simulink model "EDoS_model"  (R2020b)
settings: Solver=VariableStepAuto  StartTime=0.0  StopTime=200000  RelTol=1e-3
values from neighbouring files (symbols this model uses):
  attackRate = 0    [init_model.m]
  initialLoopWaitTime = 1000    [init_model.m]    (also in plot_results.m = 50)
  lowerUtilThreshold = 50    [init_model.m]    (also in plot_results.m)
  maxCores = 35    [init_model.m]    (also in plot_results.m)
  routineRate = 4    [init_model.m]    (also in plot_results.m)
  scalingLoopDelay = 500    [init_model.m]    (also in plot_results.m = 5)
  scalingStep = 2    [init_model.m]    (also in plot_results.m)
  upperUtilThreshold = 80    [init_model.m]    (also in plot_results.m)
undefined symbols (not defined in the file or in its folder): m, n
libraries: simulink x2
(part 2 of 3)

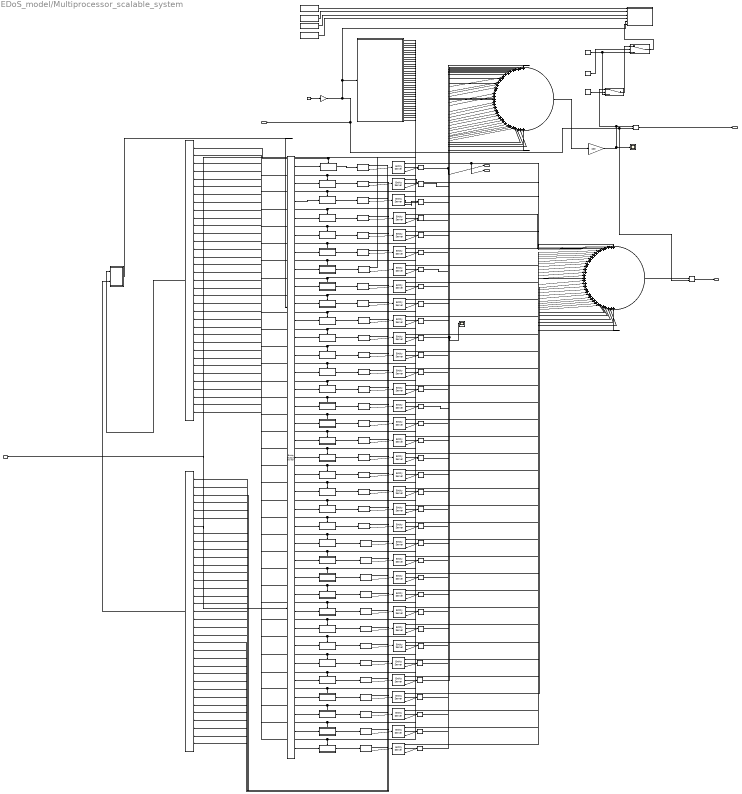
== system EDoS_model/Multiprocessor_scalable_system ==
  In1 : Inport
  Balancer : Subsystem
  Blocker : Subsystem
      settings: PortSchema="{\"entries\":[{\"content\":{\"sides\":[{\"content\":{\"connectorIds\":[\"In1\"]},\"type\":\"ConnectorPlacement.EquallySpacedRectSide\",\"uuid\":\"22857888-3c5c-4d01-b6fe-cd28fcf3e26a\"},{\"content\":{\"connectorIds\":[\"Out1\"],\"side\":\"RIGHT\"},\"type\":\"ConnectorPlacement.EquallySpacedRectSide\",\"uuid\":\"96f331b9-a29b-4997-ac5d-363cc8c82408\"},{\"content\":{\"connectorIds\":[\"In2\"],\"side\":\"TOP\"},\"type\":\"ConnectorPlacement.EquallySpacedRectSide\",\"uuid\":\"a53d43ab-ab12-479d-a738-753383dbd2f4\"},{\"content\":{\"connectorIds\":[],\"side\":\"HIDDEN\"},\"type\":\"ConnectorPlacement.EquallySpacedRectSide\",\"uuid\":\"fd9f22b1-3292-4974-90d3-70a5045257e9\"}]},\"type\":\"ConnectorPlacement.EquallySpacedConnector\",\"uuid\":\"b457ec3b-3668-4afe-a989-4fa0f92502cf\"}],\"packageUris\":[\"http://schema.mathworks.com/mf0/Connector/R2020b\"],\"version\":\"1.0\"}"
  Blocker1 : Subsystem
      settings: PortSchema="{\"entries\":[{\"content\":{\"sides\":[{\"content\":{\"connectorIds\":[\"In1\"]},\"type\":\"ConnectorPlacement.EquallySpacedRectSide\",\"uuid\":\"22857888-3c5c-4d01-b6fe-cd28fcf3e26a\"},{\"content\":{\"connectorIds\":[\"Out1\"],\"side\":\"RIGHT\"},\"type\":\"ConnectorPlacement.EquallySpacedRectSide\",\"uuid\":\"96f331b9-a29b-4997-ac5d-363cc8c82408\"},{\"content\":{\"connectorIds\":[\"In2\"],\"side\":\"TOP\"},\"type\":\"ConnectorPlacement.EquallySpacedRectSide\",\"uuid\":\"a53d43ab-ab12-479d-a738-753383dbd2f4\"},{\"content\":{\"connectorIds\":[],\"side\":\"HIDDEN\"},\"type\":\"ConnectorPlacement.EquallySpacedRectSide\",\"uuid\":\"fd9f22b1-3292-4974-90d3-70a5045257e9\"}]},\"type\":\"ConnectorPlacement.EquallySpacedConnector\",\"uuid\":\"b457ec3b-3668-4afe-a989-4fa0f92502cf\"}],\"packageUris\":[\"http://schema.mathworks.com/mf0/Connector/R2020b\"],\"version\":\"1.0\"}"
  Blocker10 : Subsystem
      settings: PortSchema="{\"entries\":[{\"content\":{\"sides\":[{\"content\":{\"connectorIds\":[\"In1\"]},\"type\":\"ConnectorPlacement.EquallySpacedRectSide\",\"uuid\":\"22857888-3c5c-4d01-b6fe-cd28fcf3e26a\"},{\"content\":{\"connectorIds\":[\"Out1\"],\"side\":\"RIGHT\"},\"type\":\"ConnectorPlacement.EquallySpacedRectSide\",\"uuid\":\"96f331b9-a29b-4997-ac5d-363cc8c82408\"},{\"content\":{\"connectorIds\":[\"In2\"],\"side\":\"TOP\"},\"type\":\"ConnectorPlacement.EquallySpacedRectSide\",\"uuid\":\"a53d43ab-ab12-479d-a738-753383dbd2f4\"},{\"content\":{\"connectorIds\":[],\"side\":\"HIDDEN\"},\"type\":\"ConnectorPlacement.EquallySpacedRectSide\",\"uuid\":\"fd9f22b1-3292-4974-90d3-70a5045257e9\"}]},\"type\":\"ConnectorPlacement.EquallySpacedConnector\",\"uuid\":\"b457ec3b-3668-4afe-a989-4fa0f92502cf\"}],\"packageUris\":[\"http://schema.mathworks.com/mf0/Connector/R2020b\"],\"version\":\"1.0\"}"
  Blocker11 : Subsystem
      settings: PortSchema="{\"entries\":[{\"content\":{\"sides\":[{\"content\":{\"connectorIds\":[\"In1\"]},\"type\":\"ConnectorPlacement.EquallySpacedRectSide\",\"uuid\":\"22857888-3c5c-4d01-b6fe-cd28fcf3e26a\"},{\"content\":{\"connectorIds\":[\"Out1\"],\"side\":\"RIGHT\"},\"type\":\"ConnectorPlacement.EquallySpacedRectSide\",\"uuid\":\"96f331b9-a29b-4997-ac5d-363cc8c82408\"},{\"content\":{\"connectorIds\":[\"In2\"],\"side\":\"TOP\"},\"type\":\"ConnectorPlacement.EquallySpacedRectSide\",\"uuid\":\"a53d43ab-ab12-479d-a738-753383dbd2f4\"},{\"content\":{\"connectorIds\":[],\"side\":\"HIDDEN\"},\"type\":\"ConnectorPlacement.EquallySpacedRectSide\",\"uuid\":\"fd9f22b1-3292-4974-90d3-70a5045257e9\"}]},\"type\":\"ConnectorPlacement.EquallySpacedConnector\",\"uuid\":\"b457ec3b-3668-4afe-a989-4fa0f92502cf\"}],\"packageUris\":[\"http://schema.mathworks.com/mf0/Connector/R2020b\"],\"version\":\"1.0\"}"
  Blocker12 : Subsystem
      settings: PortSchema="{\"entries\":[{\"content\":{\"sides\":[{\"content\":{\"connectorIds\":[\"In1\"]},\"type\":\"ConnectorPlacement.EquallySpacedRectSide\",\"uuid\":\"22857888-3c5c-4d01-b6fe-cd28fcf3e26a\"},{\"content\":{\"connectorIds\":[\"Out1\"],\"side\":\"RIGHT\"},\"type\":\"ConnectorPlacement.EquallySpacedRectSide\",\"uuid\":\"96f331b9-a29b-4997-ac5d-363cc8c82408\"},{\"content\":{\"connectorIds\":[\"In2\"],\"side\":\"TOP\"},\"type\":\"ConnectorPlacement.EquallySpacedRectSide\",\"uuid\":\"a53d43ab-ab12-479d-a738-753383dbd2f4\"},{\"content\":{\"connectorIds\":[],\"side\":\"HIDDEN\"},\"type\":\"ConnectorPlacement.EquallySpacedRectSide\",\"uuid\":\"fd9f22b1-3292-4974-90d3-70a5045257e9\"}]},\"type\":\"ConnectorPlacement.EquallySpacedConnector\",\"uuid\":\"b457ec3b-3668-4afe-a989-4fa0f92502cf\"}],\"packageUris\":[\"http://schema.mathworks.com/mf0/Connector/R2020b\"],\"version\":\"1.0\"}"
  Blocker13 : Subsystem
      settings: PortSchema="{\"entries\":[{\"content\":{\"sides\":[{\"content\":{\"connectorIds\":[\"In1\"]},\"type\":\"ConnectorPlacement.EquallySpacedRectSide\",\"uuid\":\"22857888-3c5c-4d01-b6fe-cd28fcf3e26a\"},{\"content\":{\"connectorIds\":[\"Out1\"],\"side\":\"RIGHT\"},\"type\":\"ConnectorPlacement.EquallySpacedRectSide\",\"uuid\":\"96f331b9-a29b-4997-ac5d-363cc8c82408\"},{\"content\":{\"connectorIds\":[\"In2\"],\"side\":\"TOP\"},\"type\":\"ConnectorPlacement.EquallySpacedRectSide\",\"uuid\":\"a53d43ab-ab12-479d-a738-753383dbd2f4\"},{\"content\":{\"connectorIds\":[],\"side\":\"HIDDEN\"},\"type\":\"ConnectorPlacement.EquallySpacedRectSide\",\"uuid\":\"fd9f22b1-3292-4974-90d3-70a5045257e9\"}]},\"type\":\"ConnectorPlacement.EquallySpacedConnector\",\"uuid\":\"b457ec3b-3668-4afe-a989-4fa0f92502cf\"}],\"packageUris\":[\"http://schema.mathworks.com/mf0/Connector/R2020b\"],\"version\":\"1.0\"}"
  Blocker14 : Subsystem
      settings: PortSchema="{\"entries\":[{\"content\":{\"sides\":[{\"content\":{\"connectorIds\":[\"In1\"]},\"type\":\"ConnectorPlacement.EquallySpacedRectSide\",\"uuid\":\"22857888-3c5c-4d01-b6fe-cd28fcf3e26a\"},{\"content\":{\"connectorIds\":[\"Out1\"],\"side\":\"RIGHT\"},\"type\":\"ConnectorPlacement.EquallySpacedRectSide\",\"uuid\":\"96f331b9-a29b-4997-ac5d-363cc8c82408\"},{\"content\":{\"connectorIds\":[\"In2\"],\"side\":\"TOP\"},\"type\":\"ConnectorPlacement.EquallySpacedRectSide\",\"uuid\":\"a53d43ab-ab12-479d-a738-753383dbd2f4\"},{\"content\":{\"connectorIds\":[],\"side\":\"HIDDEN\"},\"type\":\"ConnectorPlacement.EquallySpacedRectSide\",\"uuid\":\"fd9f22b1-3292-4974-90d3-70a5045257e9\"}]},\"type\":\"ConnectorPlacement.EquallySpacedConnector\",\"uuid\":\"b457ec3b-3668-4afe-a989-4fa0f92502cf\"}],\"packageUris\":[\"http://schema.mathworks.com/mf0/Connector/R2020b\"],\"version\":\"1.0\"}"
  Blocker15 : Subsystem
      settings: PortSchema="{\"entries\":[{\"content\":{\"sides\":[{\"content\":{\"connectorIds\":[\"In1\"]},\"type\":\"ConnectorPlacement.EquallySpacedRectSide\",\"uuid\":\"22857888-3c5c-4d01-b6fe-cd28fcf3e26a\"},{\"content\":{\"connectorIds\":[\"Out1\"],\"side\":\"RIGHT\"},\"type\":\"ConnectorPlacement.EquallySpacedRectSide\",\"uuid\":\"96f331b9-a29b-4997-ac5d-363cc8c82408\"},{\"content\":{\"connectorIds\":[\"In2\"],\"side\":\"TOP\"},\"type\":\"ConnectorPlacement.EquallySpacedRectSide\",\"uuid\":\"a53d43ab-ab12-479d-a738-753383dbd2f4\"},{\"content\":{\"connectorIds\":[],\"side\":\"HIDDEN\"},\"type\":\"ConnectorPlacement.EquallySpacedRectSide\",\"uuid\":\"fd9f22b1-3292-4974-90d3-70a5045257e9\"}]},\"type\":\"ConnectorPlacement.EquallySpacedConnector\",\"uuid\":\"b457ec3b-3668-4afe-a989-4fa0f92502cf\"}],\"packageUris\":[\"http://schema.mathworks.com/mf0/Connector/R2020b\"],\"version\":\"1.0\"}"
  Blocker16 : Subsystem
      settings: PortSchema="{\"entries\":[{\"content\":{\"sides\":[{\"content\":{\"connectorIds\":[\"In1\"]},\"type\":\"ConnectorPlacement.EquallySpacedRectSide\",\"uuid\":\"22857888-3c5c-4d01-b6fe-cd28fcf3e26a\"},{\"content\":{\"connectorIds\":[\"Out1\"],\"side\":\"RIGHT\"},\"type\":\"ConnectorPlacement.EquallySpacedRectSide\",\"uuid\":\"96f331b9-a29b-4997-ac5d-363cc8c82408\"},{\"content\":{\"connectorIds\":[\"In2\"],\"side\":\"TOP\"},\"type\":\"ConnectorPlacement.EquallySpacedRectSide\",\"uuid\":\"a53d43ab-ab12-479d-a738-753383dbd2f4\"},{\"content\":{\"connectorIds\":[],\"side\":\"HIDDEN\"},\"type\":\"ConnectorPlacement.EquallySpacedRectSide\",\"uuid\":\"fd9f22b1-3292-4974-90d3-70a5045257e9\"}]},\"type\":\"ConnectorPlacement.EquallySpacedConnector\",\"uuid\":\"b457ec3b-3668-4afe-a989-4fa0f92502cf\"}],\"packageUris\":[\"http://schema.mathworks.com/mf0/Connector/R2020b\"],\"version\":\"1.0\"}"
  Blocker17 : Subsystem
      settings: PortSchema="{\"entries\":[{\"content\":{\"sides\":[{\"content\":{\"connectorIds\":[\"In1\"]},\"type\":\"ConnectorPlacement.EquallySpacedRectSide\",\"uuid\":\"22857888-3c5c-4d01-b6fe-cd28fcf3e26a\"},{\"content\":{\"connectorIds\":[\"Out1\"],\"side\":\"RIGHT\"},\"type\":\"ConnectorPlacement.EquallySpacedRectSide\",\"uuid\":\"96f331b9-a29b-4997-ac5d-363cc8c82408\"},{\"content\":{\"connectorIds\":[\"In2\"],\"side\":\"TOP\"},\"type\":\"ConnectorPlacement.EquallySpacedRectSide\",\"uuid\":\"a53d43ab-ab12-479d-a738-753383dbd2f4\"},{\"content\":{\"connectorIds\":[],\"side\":\"HIDDEN\"},\"type\":\"ConnectorPlacement.EquallySpacedRectSide\",\"uuid\":\"fd9f22b1-3292-4974-90d3-70a5045257e9\"}]},\"type\":\"ConnectorPlacement.EquallySpacedConnector\",\"uuid\":\"b457ec3b-3668-4afe-a989-4fa0f92502cf\"}],\"packageUris\":[\"http://schema.mathworks.com/mf0/Connector/R2020b\"],\"version\":\"1.0\"}"
  Blocker18 : Subsystem
      settings: PortSchema="{\"entries\":[{\"content\":{\"sides\":[{\"content\":{\"connectorIds\":[\"In1\"]},\"type\":\"ConnectorPlacement.EquallySpacedRectSide\",\"uuid\":\"22857888-3c5c-4d01-b6fe-cd28fcf3e26a\"},{\"content\":{\"connectorIds\":[\"Out1\"],\"side\":\"RIGHT\"},\"type\":\"ConnectorPlacement.EquallySpacedRectSide\",\"uuid\":\"96f331b9-a29b-4997-ac5d-363cc8c82408\"},{\"content\":{\"connectorIds\":[\"In2\"],\"side\":\"TOP\"},\"type\":\"ConnectorPlacement.EquallySpacedRectSide\",\"uuid\":\"a53d43ab-ab12-479d-a738-753383dbd2f4\"},{\"content\":{\"connectorIds\":[],\"side\":\"HIDDEN\"},\"type\":\"ConnectorPlacement.EquallySpacedRectSide\",\"uuid\":\"fd9f22b1-3292-4974-90d3-70a5045257e9\"}]},\"type\":\"ConnectorPlacement.EquallySpacedConnector\",\"uuid\":\"b457ec3b-3668-4afe-a989-4fa0f92502cf\"}],\"packageUris\":[\"http://schema.mathworks.com/mf0/Connector/R2020b\"],\"version\":\"1.0\"}"
  Blocker19 : Subsystem
      settings: PortSchema="{\"entries\":[{\"content\":{\"sides\":[{\"content\":{\"connectorIds\":[\"In1\"]},\"type\":\"ConnectorPlacement.EquallySpacedRectSide\",\"uuid\":\"22857888-3c5c-4d01-b6fe-cd28fcf3e26a\"},{\"content\":{\"connectorIds\":[\"Out1\"],\"side\":\"RIGHT\"},\"type\":\"ConnectorPlacement.EquallySpacedRectSide\",\"uuid\":\"96f331b9-a29b-4997-ac5d-363cc8c82408\"},{\"content\":{\"connectorIds\":[\"In2\"],\"side\":\"TOP\"},\"type\":\"ConnectorPlacement.EquallySpacedRectSide\",\"uuid\":\"a53d43ab-ab12-479d-a738-753383dbd2f4\"},{\"content\":{\"connectorIds\":[],\"side\":\"HIDDEN\"},\"type\":\"ConnectorPlacement.EquallySpacedRectSide\",\"uuid\":\"fd9f22b1-3292-4974-90d3-70a5045257e9\"}]},\"type\":\"ConnectorPlacement.EquallySpacedConnector\",\"uuid\":\"b457ec3b-3668-4afe-a989-4fa0f92502cf\"}],\"packageUris\":[\"http://schema.mathworks.com/mf0/Connector/R2020b\"],\"version\":\"1.0\"}"
  Blocker2 : Subsystem
      settings: PortSchema="{\"entries\":[{\"content\":{\"sides\":[{\"content\":{\"connectorIds\":[\"In1\"]},\"type\":\"ConnectorPlacement.EquallySpacedRectSide\",\"uuid\":\"22857888-3c5c-4d01-b6fe-cd28fcf3e26a\"},{\"content\":{\"connectorIds\":[\"Out1\"],\"side\":\"RIGHT\"},\"type\":\"ConnectorPlacement.EquallySpacedRectSide\",\"uuid\":\"96f331b9-a29b-4997-ac5d-363cc8c82408\"},{\"content\":{\"connectorIds\":[\"In2\"],\"side\":\"TOP\"},\"type\":\"ConnectorPlacement.EquallySpacedRectSide\",\"uuid\":\"a53d43ab-ab12-479d-a738-753383dbd2f4\"},{\"content\":{\"connectorIds\":[],\"side\":\"HIDDEN\"},\"type\":\"ConnectorPlacement.EquallySpacedRectSide\",\"uuid\":\"fd9f22b1-3292-4974-90d3-70a5045257e9\"}]},\"type\":\"ConnectorPlacement.EquallySpacedConnector\",\"uuid\":\"b457ec3b-3668-4afe-a989-4fa0f92502cf\"}],\"packageUris\":[\"http://schema.mathworks.com/mf0/Connector/R2020b\"],\"version\":\"1.0\"}"
  Blocker20 : Subsystem
      settings: PortSchema="{\"entries\":[{\"content\":{\"sides\":[{\"content\":{\"connectorIds\":[\"In1\"]},\"type\":\"ConnectorPlacement.EquallySpacedRectSide\",\"uuid\":\"22857888-3c5c-4d01-b6fe-cd28fcf3e26a\"},{\"content\":{\"connectorIds\":[\"Out1\"],\"side\":\"RIGHT\"},\"type\":\"ConnectorPlacement.EquallySpacedRectSide\",\"uuid\":\"96f331b9-a29b-4997-ac5d-363cc8c82408\"},{\"content\":{\"connectorIds\":[\"In2\"],\"side\":\"TOP\"},\"type\":\"ConnectorPlacement.EquallySpacedRectSide\",\"uuid\":\"a53d43ab-ab12-479d-a738-753383dbd2f4\"},{\"content\":{\"connectorIds\":[],\"side\":\"HIDDEN\"},\"type\":\"ConnectorPlacement.EquallySpacedRectSide\",\"uuid\":\"fd9f22b1-3292-4974-90d3-70a5045257e9\"}]},\"type\":\"ConnectorPlacement.EquallySpacedConnector\",\"uuid\":\"b457ec3b-3668-4afe-a989-4fa0f92502cf\"}],\"packageUris\":[\"http://schema.mathworks.com/mf0/Connector/R2020b\"],\"version\":\"1.0\"}"
  Blocker21 : Subsystem
      settings: PortSchema="{\"entries\":[{\"content\":{\"sides\":[{\"content\":{\"connectorIds\":[\"In1\"]},\"type\":\"ConnectorPlacement.EquallySpacedRectSide\",\"uuid\":\"22857888-3c5c-4d01-b6fe-cd28fcf3e26a\"},{\"content\":{\"connectorIds\":[\"Out1\"],\"side\":\"RIGHT\"},\"type\":\"ConnectorPlacement.EquallySpacedRectSide\",\"uuid\":\"96f331b9-a29b-4997-ac5d-363cc8c82408\"},{\"content\":{\"connectorIds\":[\"In2\"],\"side\":\"TOP\"},\"type\":\"ConnectorPlacement.EquallySpacedRectSide\",\"uuid\":\"a53d43ab-ab12-479d-a738-753383dbd2f4\"},{\"content\":{\"connectorIds\":[],\"side\":\"HIDDEN\"},\"type\":\"ConnectorPlacement.EquallySpacedRectSide\",\"uuid\":\"fd9f22b1-3292-4974-90d3-70a5045257e9\"}]},\"type\":\"ConnectorPlacement.EquallySpacedConnector\",\"uuid\":\"b457ec3b-3668-4afe-a989-4fa0f92502cf\"}],\"packageUris\":[\"http://schema.mathworks.com/mf0/Connector/R2020b\"],\"version\":\"1.0\"}"
  Blocker22 : Subsystem
      settings: PortSchema="{\"entries\":[{\"content\":{\"sides\":[{\"content\":{\"connectorIds\":[\"In1\"]},\"type\":\"ConnectorPlacement.EquallySpacedRectSide\",\"uuid\":\"22857888-3c5c-4d01-b6fe-cd28fcf3e26a\"},{\"content\":{\"connectorIds\":[\"Out1\"],\"side\":\"RIGHT\"},\"type\":\"ConnectorPlacement.EquallySpacedRectSide\",\"uuid\":\"96f331b9-a29b-4997-ac5d-363cc8c82408\"},{\"content\":{\"connectorIds\":[\"In2\"],\"side\":\"TOP\"},\"type\":\"ConnectorPlacement.EquallySpacedRectSide\",\"uuid\":\"a53d43ab-ab12-479d-a738-753383dbd2f4\"},{\"content\":{\"connectorIds\":[],\"side\":\"HIDDEN\"},\"type\":\"ConnectorPlacement.EquallySpacedRectSide\",\"uuid\":\"fd9f22b1-3292-4974-90d3-70a5045257e9\"}]},\"type\":\"ConnectorPlacement.EquallySpacedConnector\",\"uuid\":\"b457ec3b-3668-4afe-a989-4fa0f92502cf\"}],\"packageUris\":[\"http://schema.mathworks.com/mf0/Connector/R2020b\"],\"version\":\"1.0\"}"
  Blocker23 : Subsystem
      settings: PortSchema="{\"entries\":[{\"content\":{\"sides\":[{\"content\":{\"connectorIds\":[\"In1\"]},\"type\":\"ConnectorPlacement.EquallySpacedRectSide\",\"uuid\":\"22857888-3c5c-4d01-b6fe-cd28fcf3e26a\"},{\"content\":{\"connectorIds\":[\"Out1\"],\"side\":\"RIGHT\"},\"type\":\"ConnectorPlacement.EquallySpacedRectSide\",\"uuid\":\"96f331b9-a29b-4997-ac5d-363cc8c82408\"},{\"content\":{\"connectorIds\":[\"In2\"],\"side\":\"TOP\"},\"type\":\"ConnectorPlacement.EquallySpacedRectSide\",\"uuid\":\"a53d43ab-ab12-479d-a738-753383dbd2f4\"},{\"content\":{\"connectorIds\":[],\"side\":\"HIDDEN\"},\"type\":\"ConnectorPlacement.EquallySpacedRectSide\",\"uuid\":\"fd9f22b1-3292-4974-90d3-70a5045257e9\"}]},\"type\":\"ConnectorPlacement.EquallySpacedConnector\",\"uuid\":\"b457ec3b-3668-4afe-a989-4fa0f92502cf\"}],\"packageUris\":[\"http://schema.mathworks.com/mf0/Connector/R2020b\"],\"version\":\"1.0\"}"
  Blocker24 : Subsystem
      settings: PortSchema="{\"entries\":[{\"content\":{\"sides\":[{\"content\":{\"connectorIds\":[\"In1\"]},\"type\":\"ConnectorPlacement.EquallySpacedRectSide\",\"uuid\":\"22857888-3c5c-4d01-b6fe-cd28fcf3e26a\"},{\"content\":{\"connectorIds\":[\"Out1\"],\"side\":\"RIGHT\"},\"type\":\"ConnectorPlacement.EquallySpacedRectSide\",\"uuid\":\"96f331b9-a29b-4997-ac5d-363cc8c82408\"},{\"content\":{\"connectorIds\":[\"In2\"],\"side\":\"TOP\"},\"type\":\"ConnectorPlacement.EquallySpacedRectSide\",\"uuid\":\"a53d43ab-ab12-479d-a738-753383dbd2f4\"},{\"content\":{\"connectorIds\":[],\"side\":\"HIDDEN\"},\"type\":\"ConnectorPlacement.EquallySpacedRectSide\",\"uuid\":\"fd9f22b1-3292-4974-90d3-70a5045257e9\"}]},\"type\":\"ConnectorPlacement.EquallySpacedConnector\",\"uuid\":\"b457ec3b-3668-4afe-a989-4fa0f92502cf\"}],\"packageUris\":[\"http://schema.mathworks.com/mf0/Connector/R2020b\"],\"version\":\"1.0\"}"
  Blocker25 : Subsystem
      settings: PortSchema="{\"entries\":[{\"content\":{\"sides\":[{\"content\":{\"connectorIds\":[\"In1\"]},\"type\":\"ConnectorPlacement.EquallySpacedRectSide\",\"uuid\":\"22857888-3c5c-4d01-b6fe-cd28fcf3e26a\"},{\"content\":{\"connectorIds\":[\"Out1\"],\"side\":\"RIGHT\"},\"type\":\"ConnectorPlacement.EquallySpacedRectSide\",\"uuid\":\"96f331b9-a29b-4997-ac5d-363cc8c82408\"},{\"content\":{\"connectorIds\":[\"In2\"],\"side\":\"TOP\"},\"type\":\"ConnectorPlacement.EquallySpacedRectSide\",\"uuid\":\"a53d43ab-ab12-479d-a738-753383dbd2f4\"},{\"content\":{\"connectorIds\":[],\"side\":\"HIDDEN\"},\"type\":\"ConnectorPlacement.EquallySpacedRectSide\",\"uuid\":\"fd9f22b1-3292-4974-90d3-70a5045257e9\"}]},\"type\":\"ConnectorPlacement.EquallySpacedConnector\",\"uuid\":\"b457ec3b-3668-4afe-a989-4fa0f92502cf\"}],\"packageUris\":[\"http://schema.mathworks.com/mf0/Connector/R2020b\"],\"version\":\"1.0\"}"
  Blocker26 : Subsystem
      settings: PortSchema="{\"entries\":[{\"content\":{\"sides\":[{\"content\":{\"connectorIds\":[\"In1\"]},\"type\":\"ConnectorPlacement.EquallySpacedRectSide\",\"uuid\":\"22857888-3c5c-4d01-b6fe-cd28fcf3e26a\"},{\"content\":{\"connectorIds\":[\"Out1\"],\"side\":\"RIGHT\"},\"type\":\"ConnectorPlacement.EquallySpacedRectSide\",\"uuid\":\"96f331b9-a29b-4997-ac5d-363cc8c82408\"},{\"content\":{\"connectorIds\":[\"In2\"],\"side\":\"TOP\"},\"type\":\"ConnectorPlacement.EquallySpacedRectSide\",\"uuid\":\"a53d43ab-ab12-479d-a738-753383dbd2f4\"},{\"content\":{\"connectorIds\":[],\"side\":\"HIDDEN\"},\"type\":\"ConnectorPlacement.EquallySpacedRectSide\",\"uuid\":\"fd9f22b1-3292-4974-90d3-70a5045257e9\"}]},\"type\":\"ConnectorPlacement.EquallySpacedConnector\",\"uuid\":\"b457ec3b-3668-4afe-a989-4fa0f92502cf\"}],\"packageUris\":[\"http://schema.mathworks.com/mf0/Connector/R2020b\"],\"version\":\"1.0\"}"
  Blocker27 : Subsystem
      settings: PortSchema="{\"entries\":[{\"content\":{\"sides\":[{\"content\":{\"connectorIds\":[\"In1\"]},\"type\":\"ConnectorPlacement.EquallySpacedRectSide\",\"uuid\":\"22857888-3c5c-4d01-b6fe-cd28fcf3e26a\"},{\"content\":{\"connectorIds\":[\"Out1\"],\"side\":\"RIGHT\"},\"type\":\"ConnectorPlacement.EquallySpacedRectSide\",\"uuid\":\"96f331b9-a29b-4997-ac5d-363cc8c82408\"},{\"content\":{\"connectorIds\":[\"In2\"],\"side\":\"TOP\"},\"type\":\"ConnectorPlacement.EquallySpacedRectSide\",\"uuid\":\"a53d43ab-ab12-479d-a738-753383dbd2f4\"},{\"content\":{\"connectorIds\":[],\"side\":\"HIDDEN\"},\"type\":\"ConnectorPlacement.EquallySpacedRectSide\",\"uuid\":\"fd9f22b1-3292-4974-90d3-70a5045257e9\"}]},\"type\":\"ConnectorPlacement.EquallySpacedConnector\",\"uuid\":\"b457ec3b-3668-4afe-a989-4fa0f92502cf\"}],\"packageUris\":[\"http://schema.mathworks.com/mf0/Connector/R2020b\"],\"version\":\"1.0\"}"
  Blocker28 : Subsystem
      settings: PortSchema="{\"entries\":[{\"content\":{\"sides\":[{\"content\":{\"connectorIds\":[\"In1\"]},\"type\":\"ConnectorPlacement.EquallySpacedRectSide\",\"uuid\":\"22857888-3c5c-4d01-b6fe-cd28fcf3e26a\"},{\"content\":{\"connectorIds\":[\"Out1\"],\"side\":\"RIGHT\"},\"type\":\"ConnectorPlacement.EquallySpacedRectSide\",\"uuid\":\"96f331b9-a29b-4997-ac5d-363cc8c82408\"},{\"content\":{\"connectorIds\":[\"In2\"],\"side\":\"TOP\"},\"type\":\"ConnectorPlacement.EquallySpacedRectSide\",\"uuid\":\"a53d43ab-ab12-479d-a738-753383dbd2f4\"},{\"content\":{\"connectorIds\":[],\"side\":\"HIDDEN\"},\"type\":\"ConnectorPlacement.EquallySpacedRectSide\",\"uuid\":\"fd9f22b1-3292-4974-90d3-70a5045257e9\"}]},\"type\":\"ConnectorPlacement.EquallySpacedConnector\",\"uuid\":\"b457ec3b-3668-4afe-a989-4fa0f92502cf\"}],\"packageUris\":[\"http://schema.mathworks.com/mf0/Connector/R2020b\"],\"version\":\"1.0\"}"
  Blocker29 : Subsystem
      settings: PortSchema="{\"entries\":[{\"content\":{\"sides\":[{\"content\":{\"connectorIds\":[\"In1\"]},\"type\":\"ConnectorPlacement.EquallySpacedRectSide\",\"uuid\":\"22857888-3c5c-4d01-b6fe-cd28fcf3e26a\"},{\"content\":{\"connectorIds\":[\"Out1\"],\"side\":\"RIGHT\"},\"type\":\"ConnectorPlacement.EquallySpacedRectSide\",\"uuid\":\"96f331b9-a29b-4997-ac5d-363cc8c82408\"},{\"content\":{\"connectorIds\":[\"In2\"],\"side\":\"TOP\"},\"type\":\"ConnectorPlacement.EquallySpacedRectSide\",\"uuid\":\"a53d43ab-ab12-479d-a738-753383dbd2f4\"},{\"content\":{\"connectorIds\":[],\"side\":\"HIDDEN\"},\"type\":\"ConnectorPlacement.EquallySpacedRectSide\",\"uuid\":\"fd9f22b1-3292-4974-90d3-70a5045257e9\"}]},\"type\":\"ConnectorPlacement.EquallySpacedConnector\",\"uuid\":\"b457ec3b-3668-4afe-a989-4fa0f92502cf\"}],\"packageUris\":[\"http://schema.mathworks.com/mf0/Connector/R2020b\"],\"version\":\"1.0\"}"
  Blocker3 : Subsystem
      settings: PortSchema="{\"entries\":[{\"content\":{\"sides\":[{\"content\":{\"connectorIds\":[\"In1\"]},\"type\":\"ConnectorPlacement.EquallySpacedRectSide\",\"uuid\":\"22857888-3c5c-4d01-b6fe-cd28fcf3e26a\"},{\"content\":{\"connectorIds\":[\"Out1\"],\"side\":\"RIGHT\"},\"type\":\"ConnectorPlacement.EquallySpacedRectSide\",\"uuid\":\"96f331b9-a29b-4997-ac5d-363cc8c82408\"},{\"content\":{\"connectorIds\":[\"In2\"],\"side\":\"TOP\"},\"type\":\"ConnectorPlacement.EquallySpacedRectSide\",\"uuid\":\"a53d43ab-ab12-479d-a738-753383dbd2f4\"},{\"content\":{\"connectorIds\":[],\"side\":\"HIDDEN\"},\"type\":\"ConnectorPlacement.EquallySpacedRectSide\",\"uuid\":\"fd9f22b1-3292-4974-90d3-70a5045257e9\"}]},\"type\":\"ConnectorPlacement.EquallySpacedConnector\",\"uuid\":\"b457ec3b-3668-4afe-a989-4fa0f92502cf\"}],\"packageUris\":[\"http://schema.mathworks.com/mf0/Connector/R2020b\"],\"version\":\"1.0\"}"
  Blocker30 : Subsystem
      settings: PortSchema="{\"entries\":[{\"content\":{\"sides\":[{\"content\":{\"connectorIds\":[\"In1\"]},\"type\":\"ConnectorPlacement.EquallySpacedRectSide\",\"uuid\":\"22857888-3c5c-4d01-b6fe-cd28fcf3e26a\"},{\"content\":{\"connectorIds\":[\"Out1\"],\"side\":\"RIGHT\"},\"type\":\"ConnectorPlacement.EquallySpacedRectSide\",\"uuid\":\"96f331b9-a29b-4997-ac5d-363cc8c82408\"},{\"content\":{\"connectorIds\":[\"In2\"],\"side\":\"TOP\"},\"type\":\"ConnectorPlacement.EquallySpacedRectSide\",\"uuid\":\"a53d43ab-ab12-479d-a738-753383dbd2f4\"},{\"content\":{\"connectorIds\":[],\"side\":\"HIDDEN\"},\"type\":\"ConnectorPlacement.EquallySpacedRectSide\",\"uuid\":\"fd9f22b1-3292-4974-90d3-70a5045257e9\"}]},\"type\":\"ConnectorPlacement.EquallySpacedConnector\",\"uuid\":\"b457ec3b-3668-4afe-a989-4fa0f92502cf\"}],\"packageUris\":[\"http://schema.mathworks.com/mf0/Connector/R2020b\"],\"version\":\"1.0\"}"
  Blocker31 : Subsystem
      settings: PortSchema="{\"entries\":[{\"content\":{\"sides\":[{\"content\":{\"connectorIds\":[\"In1\"]},\"type\":\"ConnectorPlacement.EquallySpacedRectSide\",\"uuid\":\"22857888-3c5c-4d01-b6fe-cd28fcf3e26a\"},{\"content\":{\"connectorIds\":[\"Out1\"],\"side\":\"RIGHT\"},\"type\":\"ConnectorPlacement.EquallySpacedRectSide\",\"uuid\":\"96f331b9-a29b-4997-ac5d-363cc8c82408\"},{\"content\":{\"connectorIds\":[\"In2\"],\"side\":\"TOP\"},\"type\":\"ConnectorPlacement.EquallySpacedRectSide\",\"uuid\":\"a53d43ab-ab12-479d-a738-753383dbd2f4\"},{\"content\":{\"connectorIds\":[],\"side\":\"HIDDEN\"},\"type\":\"ConnectorPlacement.EquallySpacedRectSide\",\"uuid\":\"fd9f22b1-3292-4974-90d3-70a5045257e9\"}]},\"type\":\"ConnectorPlacement.EquallySpacedConnector\",\"uuid\":\"b457ec3b-3668-4afe-a989-4fa0f92502cf\"}],\"packageUris\":[\"http://schema.mathworks.com/mf0/Connector/R2020b\"],\"version\":\"1.0\"}"
  Blocker32 : Subsystem
      settings: PortSchema="{\"entries\":[{\"content\":{\"sides\":[{\"content\":{\"connectorIds\":[\"In1\"]},\"type\":\"ConnectorPlacement.EquallySpacedRectSide\",\"uuid\":\"22857888-3c5c-4d01-b6fe-cd28fcf3e26a\"},{\"content\":{\"connectorIds\":[\"Out1\"],\"side\":\"RIGHT\"},\"type\":\"ConnectorPlacement.EquallySpacedRectSide\",\"uuid\":\"96f331b9-a29b-4997-ac5d-363cc8c82408\"},{\"content\":{\"connectorIds\":[\"In2\"],\"side\":\"TOP\"},\"type\":\"ConnectorPlacement.EquallySpacedRectSide\",\"uuid\":\"a53d43ab-ab12-479d-a738-753383dbd2f4\"},{\"content\":{\"connectorIds\":[],\"side\":\"HIDDEN\"},\"type\":\"ConnectorPlacement.EquallySpacedRectSide\",\"uuid\":\"fd9f22b1-3292-4974-90d3-70a5045257e9\"}]},\"type\":\"ConnectorPlacement.EquallySpacedConnector\",\"uuid\":\"b457ec3b-3668-4afe-a989-4fa0f92502cf\"}],\"packageUris\":[\"http://schema.mathworks.com/mf0/Connector/R2020b\"],\"version\":\"1.0\"}"
  Blocker33 : Subsystem
      settings: PortSchema="{\"entries\":[{\"content\":{\"sides\":[{\"content\":{\"connectorIds\":[\"In1\"]},\"type\":\"ConnectorPlacement.EquallySpacedRectSide\",\"uuid\":\"22857888-3c5c-4d01-b6fe-cd28fcf3e26a\"},{\"content\":{\"connectorIds\":[\"Out1\"],\"side\":\"RIGHT\"},\"type\":\"ConnectorPlacement.EquallySpacedRectSide\",\"uuid\":\"96f331b9-a29b-4997-ac5d-363cc8c82408\"},{\"content\":{\"connectorIds\":[\"In2\"],\"side\":\"TOP\"},\"type\":\"ConnectorPlacement.EquallySpacedRectSide\",\"uuid\":\"a53d43ab-ab12-479d-a738-753383dbd2f4\"},{\"content\":{\"connectorIds\":[],\"side\":\"HIDDEN\"},\"type\":\"ConnectorPlacement.EquallySpacedRectSide\",\"uuid\":\"fd9f22b1-3292-4974-90d3-70a5045257e9\"}]},\"type\":\"ConnectorPlacement.EquallySpacedConnector\",\"uuid\":\"b457ec3b-3668-4afe-a989-4fa0f92502cf\"}],\"packageUris\":[\"http://schema.mathworks.com/mf0/Connector/R2020b\"],\"version\":\"1.0\"}"
  Blocker34 : Subsystem
      settings: PortSchema="{\"entries\":[{\"content\":{\"sides\":[{\"content\":{\"connectorIds\":[\"In1\"]},\"type\":\"ConnectorPlacement.EquallySpacedRectSide\",\"uuid\":\"22857888-3c5c-4d01-b6fe-cd28fcf3e26a\"},{\"content\":{\"connectorIds\":[\"Out1\"],\"side\":\"RIGHT\"},\"type\":\"ConnectorPlacement.EquallySpacedRectSide\",\"uuid\":\"96f331b9-a29b-4997-ac5d-363cc8c82408\"},{\"content\":{\"connectorIds\":[\"In2\"],\"side\":\"TOP\"},\"type\":\"ConnectorPlacement.EquallySpacedRectSide\",\"uuid\":\"a53d43ab-ab12-479d-a738-753383dbd2f4\"},{\"content\":{\"connectorIds\":[],\"side\":\"HIDDEN\"},\"type\":\"ConnectorPlacement.EquallySpacedRectSide\",\"uuid\":\"fd9f22b1-3292-4974-90d3-70a5045257e9\"}]},\"type\":\"ConnectorPlacement.EquallySpacedConnector\",\"uuid\":\"b457ec3b-3668-4afe-a989-4fa0f92502cf\"}],\"packageUris\":[\"http://schema.mathworks.com/mf0/Connector/R2020b\"],\"version\":\"1.0\"}"
  Blocker4 : Subsystem
      settings: PortSchema="{\"entries\":[{\"content\":{\"sides\":[{\"content\":{\"connectorIds\":[\"In1\"]},\"type\":\"ConnectorPlacement.EquallySpacedRectSide\",\"uuid\":\"22857888-3c5c-4d01-b6fe-cd28fcf3e26a\"},{\"content\":{\"connectorIds\":[\"Out1\"],\"side\":\"RIGHT\"},\"type\":\"ConnectorPlacement.EquallySpacedRectSide\",\"uuid\":\"96f331b9-a29b-4997-ac5d-363cc8c82408\"},{\"content\":{\"connectorIds\":[\"In2\"],\"side\":\"TOP\"},\"type\":\"ConnectorPlacement.EquallySpacedRectSide\",\"uuid\":\"a53d43ab-ab12-479d-a738-753383dbd2f4\"},{\"content\":{\"connectorIds\":[],\"side\":\"HIDDEN\"},\"type\":\"ConnectorPlacement.EquallySpacedRectSide\",\"uuid\":\"fd9f22b1-3292-4974-90d3-70a5045257e9\"}]},\"type\":\"ConnectorPlacement.EquallySpacedConnector\",\"uuid\":\"b457ec3b-3668-4afe-a989-4fa0f92502cf\"}],\"packageUris\":[\"http://schema.mathworks.com/mf0/Connector/R2020b\"],\"version\":\"1.0\"}"
  Blocker5 : Subsystem
      settings: PortSchema="{\"entries\":[{\"content\":{\"sides\":[{\"content\":{\"connectorIds\":[\"In1\"]},\"type\":\"ConnectorPlacement.EquallySpacedRectSide\",\"uuid\":\"22857888-3c5c-4d01-b6fe-cd28fcf3e26a\"},{\"content\":{\"connectorIds\":[\"Out1\"],\"side\":\"RIGHT\"},\"type\":\"ConnectorPlacement.EquallySpacedRectSide\",\"uuid\":\"96f331b9-a29b-4997-ac5d-363cc8c82408\"},{\"content\":{\"connectorIds\":[\"In2\"],\"side\":\"TOP\"},\"type\":\"ConnectorPlacement.EquallySpacedRectSide\",\"uuid\":\"a53d43ab-ab12-479d-a738-753383dbd2f4\"},{\"content\":{\"connectorIds\":[],\"side\":\"HIDDEN\"},\"type\":\"ConnectorPlacement.EquallySpacedRectSide\",\"uuid\":\"fd9f22b1-3292-4974-90d3-70a5045257e9\"}]},\"type\":\"ConnectorPlacement.EquallySpacedConnector\",\"uuid\":\"b457ec3b-3668-4afe-a989-4fa0f92502cf\"}],\"packageUris\":[\"http://schema.mathworks.com/mf0/Connector/R2020b\"],\"version\":\"1.0\"}"
  Blocker6 : Subsystem
      settings: PortSchema="{\"entries\":[{\"content\":{\"sides\":[{\"content\":{\"connectorIds\":[\"In1\"]},\"type\":\"ConnectorPlacement.EquallySpacedRectSide\",\"uuid\":\"22857888-3c5c-4d01-b6fe-cd28fcf3e26a\"},{\"content\":{\"connectorIds\":[\"Out1\"],\"side\":\"RIGHT\"},\"type\":\"ConnectorPlacement.EquallySpacedRectSide\",\"uuid\":\"96f331b9-a29b-4997-ac5d-363cc8c82408\"},{\"content\":{\"connectorIds\":[\"In2\"],\"side\":\"TOP\"},\"type\":\"ConnectorPlacement.EquallySpacedRectSide\",\"uuid\":\"a53d43ab-ab12-479d-a738-753383dbd2f4\"},{\"content\":{\"connectorIds\":[],\"side\":\"HIDDEN\"},\"type\":\"ConnectorPlacement.EquallySpacedRectSide\",\"uuid\":\"fd9f22b1-3292-4974-90d3-70a5045257e9\"}]},\"type\":\"ConnectorPlacement.EquallySpacedConnector\",\"uuid\":\"b457ec3b-3668-4afe-a989-4fa0f92502cf\"}],\"packageUris\":[\"http://schema.mathworks.com/mf0/Connector/R2020b\"],\"version\":\"1.0\"}"
  Blocker7 : Subsystem
      settings: PortSchema="{\"entries\":[{\"content\":{\"sides\":[{\"content\":{\"connectorIds\":[\"In1\"]},\"type\":\"ConnectorPlacement.EquallySpacedRectSide\",\"uuid\":\"22857888-3c5c-4d01-b6fe-cd28fcf3e26a\"},{\"content\":{\"connectorIds\":[\"Out1\"],\"side\":\"RIGHT\"},\"type\":\"ConnectorPlacement.EquallySpacedRectSide\",\"uuid\":\"96f331b9-a29b-4997-ac5d-363cc8c82408\"},{\"content\":{\"connectorIds\":[\"In2\"],\"side\":\"TOP\"},\"type\":\"ConnectorPlacement.EquallySpacedRectSide\",\"uuid\":\"a53d43ab-ab12-479d-a738-753383dbd2f4\"},{\"content\":{\"connectorIds\":[],\"side\":\"HIDDEN\"},\"type\":\"ConnectorPlacement.EquallySpacedRectSide\",\"uuid\":\"fd9f22b1-3292-4974-90d3-70a5045257e9\"}]},\"type\":\"ConnectorPlacement.EquallySpacedConnector\",\"uuid\":\"b457ec3b-3668-4afe-a989-4fa0f92502cf\"}],\"packageUris\":[\"http://schema.mathworks.com/mf0/Connector/R2020b\"],\"version\":\"1.0\"}"
  Blocker8 : Subsystem
      settings: PortSchema="{\"entries\":[{\"content\":{\"sides\":[{\"content\":{\"connectorIds\":[\"In1\"]},\"type\":\"ConnectorPlacement.EquallySpacedRectSide\",\"uuid\":\"22857888-3c5c-4d01-b6fe-cd28fcf3e26a\"},{\"content\":{\"connectorIds\":[\"Out1\"],\"side\":\"RIGHT\"},\"type\":\"ConnectorPlacement.EquallySpacedRectSide\",\"uuid\":\"96f331b9-a29b-4997-ac5d-363cc8c82408\"},{\"content\":{\"connectorIds\":[\"In2\"],\"side\":\"TOP\"},\"type\":\"ConnectorPlacement.EquallySpacedRectSide\",\"uuid\":\"a53d43ab-ab12-479d-a738-753383dbd2f4\"},{\"content\":{\"connectorIds\":[],\"side\":\"HIDDEN\"},\"type\":\"ConnectorPlacement.EquallySpacedRectSide\",\"uuid\":\"fd9f22b1-3292-4974-90d3-70a5045257e9\"}]},\"type\":\"ConnectorPlacement.EquallySpacedConnector\",\"uuid\":\"b457ec3b-3668-4afe-a989-4fa0f92502cf\"}],\"packageUris\":[\"http://schema.mathworks.com/mf0/Connector/R2020b\"],\"version\":\"1.0\"}"
  Blocker9 : Subsystem
      settings: PortSchema="{\"entries\":[{\"content\":{\"sides\":[{\"content\":{\"connectorIds\":[\"In1\"]},\"type\":\"ConnectorPlacement.EquallySpacedRectSide\",\"uuid\":\"22857888-3c5c-4d01-b6fe-cd28fcf3e26a\"},{\"content\":{\"connectorIds\":[\"Out1\"],\"side\":\"RIGHT\"},\"type\":\"ConnectorPlacement.EquallySpacedRectSide\",\"uuid\":\"96f331b9-a29b-4997-ac5d-363cc8c82408\"},{\"content\":{\"connectorIds\":[\"In2\"],\"side\":\"TOP\"},\"type\":\"ConnectorPlacement.EquallySpacedRectSide\",\"uuid\":\"a53d43ab-ab12-479d-a738-753383dbd2f4\"},{\"content\":{\"connectorIds\":[],\"side\":\"HIDDEN\"},\"type\":\"ConnectorPlacement.EquallySpacedRectSide\",\"uuid\":\"fd9f22b1-3292-4974-90d3-70a5045257e9\"}]},\"type\":\"ConnectorPlacement.EquallySpacedConnector\",\"uuid\":\"b457ec3b-3668-4afe-a989-4fa0f92502cf\"}],\"packageUris\":[\"http://schema.mathworks.com/mf0/Connector/R2020b\"],\"version\":\"1.0\"}"
  Constant : Constant  SampleTime=1
  Constant1 : Constant  Value=maxCores
  Constant2 : Constant  Value=lowerUtilThreshold
  Constant3 : Constant  Value=upperUtilThreshold
  Constant4 : Constant  Value=0
  Constant5 : Constant  Value=scalingStep
  Core controller : Subsystem
  Counter Free-Running : simulink/Sources/Counter Free-Running  NumBits=16  tsamp=1
  Counter Limited : simulink/Sources/Counter Limited  uplimit=scalingLoopDelay  tsamp=1
  Divide : Product  Inputs=*/
  Divide1 : Product  Inputs=*/
  Entity Output Switch : EntityOutputSwitch  InputPortMessageModes=m,m  OutputPortMessageModes=m,m,m,m,m,m,m,m,m,m,m,m,m,m,m,m,m,m,m,m,m,m,m,m,m,m,m,m,m,m,m,m,m,m,m  NumberOutputPorts=35  SwitchingCriterion=From control port  SwitchAttributeName=Attribute1
      settings: InputPortMap=u0,u1  OutputPortMap=o0,o1,o2,o3,o4,o5,o6,o7,o8,o9,o10,o11,o12,o13,o14,o15,o16,o17,o18,o19,o20,o21,o22,o23,o24,o25,o26,o27,o28,o29,o30,o31,o32,o33,o34
  Entity Queue{,1..34} (35 alike) : Queue  InputPortMessageModes=m  OutputPortMessageModes=n,n,m  Capacity=lenOfCoreFIFO  NumberEntitiesInBlock=on  AverageWait=on
      settings: OutputPortMap=o1,o2,o5
  Entity Server : EntityServer  InputPortMessageModes=m  OutputPortMessageModes=n,n,m  Capacity=1  ServiceTimeSource=MATLAB action  ServiceTimeValue=20  ServiceTimeAttributeName=entity.ServiceTime  ServiceTimeAction=|  AverageWait=on  Utilization=on
      | c = 0.767 - 3.36/lambda;
      |     beta = pi/sqrt(3.0*lambda);
      |     alpha = beta*lambda;
      |     k = log(c) - lambda - log(beta);
      | 
      |     while true
      |         u = rand(1);
      | 	    x = (alpha - log((1.0 - u)/u))/beta;
      | 	    n = floor(x + 0.5);
      | 	    if (n < 0)
      | 		    continue;
      |         end    
      | 	    v = rand(1);
      | 	    y = alpha - beta*x;
      | 	    lhs = y + log(v/(1.0 + exp(y))^2);
      | 	    rhs = k + n*log(lambda) - log(factorial(n));
      | 	    if (lhs <= rhs)
      | 		    break;
      |         end    
      |     end  
      |     dt = n / serviceRate;
      settings: OutputPortMap=o4,o5,o9
  Entity Server1 : EntityServer  InputPortMessageModes=m  OutputPortMessageModes=n,n,m  Capacity=1  ServiceTimeSource=MATLAB action  ServiceTimeValue=20  ServiceTimeAttributeName=entity.ServiceTime  ServiceTimeAction=|  AverageWait=on  Utilization=on
      | c = 0.767 - 3.36/lambda;
      |     beta = pi/sqrt(3.0*lambda);
      |     alpha = beta*lambda;
      |     k = log(c) - lambda - log(beta);
      | 
      |     while true
      |         u = rand(1);
      | 	    x = (alpha - log((1.0 - u)/u))/beta;
      | 	    n = floor(x + 0.5);
      | 	    if (n < 0)
      | 		    continue;
      |         end    
      | 	    v = rand(1);
      | 	    y = alpha - beta*x;
      | 	    lhs = y + log(v/(1.0 + exp(y))^2);
      | 	    rhs = k + n*log(lambda) - log(factorial(n));
      | 	    if (lhs <= rhs)
      | 		    break;
      |         end    
      |     end  
      |     dt = n / serviceRate;
      settings: OutputPortMap=o4,o5,o9
  Entity Server10 : EntityServer  InputPortMessageModes=m  OutputPortMessageModes=n,n,m  Capacity=1  ServiceTimeSource=MATLAB action  ServiceTimeValue=20  ServiceTimeAttributeName=entity.ServiceTime  ServiceTimeAction=|  AverageWait=on  Utilization=on
      | c = 0.767 - 3.36/lambda;
      |     beta = pi/sqrt(3.0*lambda);
      |     alpha = beta*lambda;
      |     k = log(c) - lambda - log(beta);
      | 
      |     while true
      |         u = rand(1);
      | 	    x = (alpha - log((1.0 - u)/u))/beta;
      | 	    n = floor(x + 0.5);
      | 	    if (n < 0)
      | 		    continue;
      |         end    
      | 	    v = rand(1);
      | 	    y = alpha - beta*x;
      | 	    lhs = y + log(v/(1.0 + exp(y))^2);
      | 	    rhs = k + n*log(lambda) - log(factorial(n));
      | 	    if (lhs <= rhs)
      | 		    break;
      |         end    
      |     end  
      |     dt = n / serviceRate;
      settings: OutputPortMap=o4,o5,o9
  Entity Server11 : EntityServer  InputPortMessageModes=m  OutputPortMessageModes=n,n,m  Capacity=1  ServiceTimeSource=MATLAB action  ServiceTimeValue=20  ServiceTimeAttributeName=entity.ServiceTime  ServiceTimeAction=|  AverageWait=on  Utilization=on
      | c = 0.767 - 3.36/lambda;
      |     beta = pi/sqrt(3.0*lambda);
      |     alpha = beta*lambda;
      |     k = log(c) - lambda - log(beta);
      | 
      |     while true
      |         u = rand(1);
      | 	    x = (alpha - log((1.0 - u)/u))/beta;
      | 	    n = floor(x + 0.5);
      | 	    if (n < 0)
      | 		    continue;
      |         end    
      | 	    v = rand(1);
      | 	    y = alpha - beta*x;
      | 	    lhs = y + log(v/(1.0 + exp(y))^2);
      | 	    rhs = k + n*log(lambda) - log(factorial(n));
      | 	    if (lhs <= rhs)
      | 		    break;
      |         end    
      |     end  
      |     dt = n / serviceRate;
      settings: OutputPortMap=o4,o5,o9
  Entity Server12 : EntityServer  InputPortMessageModes=m  OutputPortMessageModes=n,n,m  Capacity=1  ServiceTimeSource=MATLAB action  ServiceTimeValue=20  ServiceTimeAttributeName=entity.ServiceTime  ServiceTimeAction=|  AverageWait=on  Utilization=on
      | c = 0.767 - 3.36/lambda;
      |     beta = pi/sqrt(3.0*lambda);
      |     alpha = beta*lambda;
      |     k = log(c) - lambda - log(beta);
      | 
      |     while true
      |         u = rand(1);
      | 	    x = (alpha - log((1.0 - u)/u))/beta;
      | 	    n = floor(x + 0.5);
      | 	    if (n < 0)
      | 		    continue;
      |         end    
      | 	    v = rand(1);
      | 	    y = alpha - beta*x;
      | 	    lhs = y + log(v/(1.0 + exp(y))^2);
      | 	    rhs = k + n*log(lambda) - log(factorial(n));
      | 	    if (lhs <= rhs)
      | 		    break;
      |         end    
      |     end  
      |     dt = n / serviceRate;
      settings: OutputPortMap=o4,o5,o9
  Entity Server13 : EntityServer  InputPortMessageModes=m  OutputPortMessageModes=n,n,m  Capacity=1  ServiceTimeSource=MATLAB action  ServiceTimeValue=20  ServiceTimeAttributeName=entity.ServiceTime  ServiceTimeAction=|  AverageWait=on  Utilization=on
      | c = 0.767 - 3.36/lambda;
      |     beta = pi/sqrt(3.0*lambda);
      |     alpha = beta*lambda;
      |     k = log(c) - lambda - log(beta);
      | 
      |     while true
      |         u = rand(1);
      | 	    x = (alpha - log((1.0 - u)/u))/beta;
      | 	    n = floor(x + 0.5);
      | 	    if (n < 0)
      | 		    continue;
      |         end    
      | 	    v = rand(1);
      | 	    y = alpha - beta*x;
      | 	    lhs = y + log(v/(1.0 + exp(y))^2);
      | 	    rhs = k + n*log(lambda) - log(factorial(n));
      | 	    if (lhs <= rhs)
      | 		    break;
      |         end    
      |     end  
      |     dt = n / serviceRate;
      settings: OutputPortMap=o4,o5,o9
  Entity Server14 : EntityServer  InputPortMessageModes=m  OutputPortMessageModes=n,n,m  Capacity=1  ServiceTimeSource=MATLAB action  ServiceTimeValue=20  ServiceTimeAttributeName=entity.ServiceTime  ServiceTimeAction=|  AverageWait=on  Utilization=on
      | c = 0.767 - 3.36/lambda;
      |     beta = pi/sqrt(3.0*lambda);
      |     alpha = beta*lambda;
      |     k = log(c) - lambda - log(beta);
      | 
      |     while true
      |         u = rand(1);
      | 	    x = (alpha - log((1.0 - u)/u))/beta;
      | 	    n = floor(x + 0.5);
      | 	    if (n < 0)
      | 		    continue;
      |         end    
      | 	    v = rand(1);
      | 	    y = alpha - beta*x;
      | 	    lhs = y + log(v/(1.0 + exp(y))^2);
      | 	    rhs = k + n*log(lambda) - log(factorial(n));
      | 	    if (lhs <= rhs)
      | 		    break;
      |         end    
      |     end  
      |     dt = n / serviceRate;
      settings: OutputPortMap=o4,o5,o9
  Entity Server15 : EntityServer  InputPortMessageModes=m  OutputPortMessageModes=n,n,m  Capacity=1  ServiceTimeSource=MATLAB action  ServiceTimeValue=20  ServiceTimeAttributeName=entity.ServiceTime  ServiceTimeAction=|  AverageWait=on  Utilization=on
      | c = 0.767 - 3.36/lambda;
      |     beta = pi/sqrt(3.0*lambda);
      |     alpha = beta*lambda;
      |     k = log(c) - lambda - log(beta);
      | 
      |     while true
      |         u = rand(1);
      | 	    x = (alpha - log((1.0 - u)/u))/beta;
      | 	    n = floor(x + 0.5);
      | 	    if (n < 0)
      | 		    continue;
      |         end    
      | 	    v = rand(1);
      | 	    y = alpha - beta*x;
      | 	    lhs = y + log(v/(1.0 + exp(y))^2);
      | 	    rhs = k + n*log(lambda) - log(factorial(n));
      | 	    if (lhs <= rhs)
      | 		    break;
      |         end    
      |     end  
      |     dt = n / serviceRate;
      settings: OutputPortMap=o4,o5,o9
  Entity Server16 : EntityServer  InputPortMessageModes=m  OutputPortMessageModes=n,n,m  Capacity=1  ServiceTimeSource=MATLAB action  ServiceTimeValue=20  ServiceTimeAttributeName=entity.ServiceTime  ServiceTimeAction=|  AverageWait=on  Utilization=on
      | c = 0.767 - 3.36/lambda;
      |     beta = pi/sqrt(3.0*lambda);
      |     alpha = beta*lambda;
      |     k = log(c) - lambda - log(beta);
      | 
      |     while true
      |         u = rand(1);
      | 	    x = (alpha - log((1.0 - u)/u))/beta;
      | 	    n = floor(x + 0.5);
      | 	    if (n < 0)
      | 		    continue;
      |         end    
      | 	    v = rand(1);
      | 	    y = alpha - beta*x;
      | 	    lhs = y + log(v/(1.0 + exp(y))^2);
      | 	    rhs = k + n*log(lambda) - log(factorial(n));
      | 	    if (lhs <= rhs)
      | 		    break;
      |         end    
      |     end  
      |     dt = n / serviceRate;
      settings: OutputPortMap=o4,o5,o9
  Entity Server17 : EntityServer  InputPortMessageModes=m  OutputPortMessageModes=n,n,m  Capacity=1  ServiceTimeSource=MATLAB action  ServiceTimeValue=20  ServiceTimeAttributeName=entity.ServiceTime  ServiceTimeAction=|  AverageWait=on  Utilization=on
      | c = 0.767 - 3.36/lambda;
      |     beta = pi/sqrt(3.0*lambda);
      |     alpha = beta*lambda;
      |     k = log(c) - lambda - log(beta);
      | 
      |     while true
      |         u = rand(1);
      | 	    x = (alpha - log((1.0 - u)/u))/beta;
      | 	    n = floor(x + 0.5);
      | 	    if (n < 0)
      | 		    continue;
      |         end    
      | 	    v = rand(1);
      | 	    y = alpha - beta*x;
      | 	    lhs = y + log(v/(1.0 + exp(y))^2);
      | 	    rhs = k + n*log(lambda) - log(factorial(n));
      | 	    if (lhs <= rhs)
      | 		    break;
      |         end    
      |     end  
      |     dt = n / serviceRate;
      settings: OutputPortMap=o4,o5,o9
  Entity Server18 : EntityServer  InputPortMessageModes=m  OutputPortMessageModes=n,n,m  Capacity=1  ServiceTimeSource=MATLAB action  ServiceTimeValue=20  ServiceTimeAttributeName=entity.ServiceTime  ServiceTimeAction=|  AverageWait=on  Utilization=on
      | c = 0.767 - 3.36/lambda;
      |     beta = pi/sqrt(3.0*lambda);
      |     alpha = beta*lambda;
      |     k = log(c) - lambda - log(beta);
      | 
      |     while true
      |         u = rand(1);
      | 	    x = (alpha - log((1.0 - u)/u))/beta;
      | 	    n = floor(x + 0.5);
      | 	    if (n < 0)
      | 		    continue;
      |         end    
      | 	    v = rand(1);
      | 	    y = alpha - beta*x;
      | 	    lhs = y + log(v/(1.0 + exp(y))^2);
      | 	    rhs = k + n*log(lambda) - log(factorial(n));
      | 	    if (lhs <= rhs)
      | 		    break;
      |         end    
      |     end  
      |     dt = n / serviceRate;
      settings: OutputPortMap=o4,o5,o9
  Entity Server19 : EntityServer  InputPortMessageModes=m  OutputPortMessageModes=n,n,m  Capacity=1  ServiceTimeSource=MATLAB action  ServiceTimeValue=20  ServiceTimeAttributeName=entity.ServiceTime  ServiceTimeAction=|  AverageWait=on  Utilization=on
      | c = 0.767 - 3.36/lambda;
      |     beta = pi/sqrt(3.0*lambda);
      |     alpha = beta*lambda;
      |     k = log(c) - lambda - log(beta);
      | 
      |     while true
      |         u = rand(1);
      | 	    x = (alpha - log((1.0 - u)/u))/beta;
      | 	    n = floor(x + 0.5);
      | 	    if (n < 0)
      | 		    continue;
      |         end    
      | 	    v = rand(1);
      | 	    y = alpha - beta*x;
      | 	    lhs = y + log(v/(1.0 + exp(y))^2);
      | 	    rhs = k + n*log(lambda) - log(factorial(n));
      | 	    if (lhs <= rhs)
      | 		    break;
      |         end    
      |     end  
      |     dt = n / serviceRate;
      settings: OutputPortMap=o4,o5,o9
  Entity Server2 : EntityServer  InputPortMessageModes=m  OutputPortMessageModes=n,n,m  Capacity=1  ServiceTimeSource=MATLAB action  ServiceTimeValue=inf  ServiceTimeAttributeName=entity.ServiceTime  ServiceTimeAction=|  AverageWait=on  Utilization=on
      | c = 0.767 - 3.36/lambda;
      |     beta = pi/sqrt(3.0*lambda);
      |     alpha = beta*lambda;
      |     k = log(c) - lambda - log(beta);
      | 
      |     while true
      |         u = rand(1);
      | 	    x = (alpha - log((1.0 - u)/u))/beta;
      | 	    n = floor(x + 0.5);
      | 	    if (n < 0)
      | 		    continue;
      |         end    
      | 	    v = rand(1);
      | 	    y = alpha - beta*x;
      | 	    lhs = y + log(v/(1.0 + exp(y))^2);
      | 	    rhs = k + n*log(lambda) - log(factorial(n));
      | 	    if (lhs <= rhs)
      | 		    break;
      |         end    
      |     end  
      |     dt = n / serviceRate;
      settings: OutputPortMap=o4,o5,o9
  Entity Server20 : EntityServer  InputPortMessageModes=m  OutputPortMessageModes=n,n,m  Capacity=1  ServiceTimeSource=MATLAB action  ServiceTimeValue=20  ServiceTimeAttributeName=entity.ServiceTime  ServiceTimeAction=|  AverageWait=on  Utilization=on
      | c = 0.767 - 3.36/lambda;
      |     beta = pi/sqrt(3.0*lambda);
      |     alpha = beta*lambda;
      |     k = log(c) - lambda - log(beta);
      | 
      |     while true
      |         u = rand(1);
      | 	    x = (alpha - log((1.0 - u)/u))/beta;
      | 	    n = floor(x + 0.5);
      | 	    if (n < 0)
      | 		    continue;
      |         end    
      | 	    v = rand(1);
      | 	    y = alpha - beta*x;
      | 	    lhs = y + log(v/(1.0 + exp(y))^2);
      | 	    rhs = k + n*log(lambda) - log(factorial(n));
      | 	    if (lhs <= rhs)
      | 		    break;
      |         end    
      |     end  
      |     dt = n / serviceRate;
      settings: OutputPortMap=o4,o5,o9
  Entity Server21 : EntityServer  InputPortMessageModes=m  OutputPortMessageModes=n,n,m  Capacity=1  ServiceTimeSource=MATLAB action  ServiceTimeValue=20  ServiceTimeAttributeName=entity.ServiceTime  ServiceTimeAction=|  AverageWait=on  Utilization=on
      | c = 0.767 - 3.36/lambda;
      |     beta = pi/sqrt(3.0*lambda);
      |     alpha = beta*lambda;
      |     k = log(c) - lambda - log(beta);
      | 
      |     while true
      |         u = rand(1);
      | 	    x = (alpha - log((1.0 - u)/u))/beta;
      | 	    n = floor(x + 0.5);
      | 	    if (n < 0)
      | 		    continue;
      |         end    
      | 	    v = rand(1);
      | 	    y = alpha - beta*x;
      | 	    lhs = y + log(v/(1.0 + exp(y))^2);
      | 	    rhs = k + n*log(lambda) - log(factorial(n));
      | 	    if (lhs <= rhs)
      | 		    break;
      |         end    
      |     end  
      |     dt = n / serviceRate;
      settings: OutputPortMap=o4,o5,o9
  Entity Server22 : EntityServer  InputPortMessageModes=m  OutputPortMessageModes=n,n,m  Capacity=1  ServiceTimeSource=MATLAB action  ServiceTimeValue=20  ServiceTimeAttributeName=entity.ServiceTime  ServiceTimeAction=|  AverageWait=on  Utilization=on
      | c = 0.767 - 3.36/lambda;
      |     beta = pi/sqrt(3.0*lambda);
      |     alpha = beta*lambda;
      |     k = log(c) - lambda - log(beta);
      | 
      |     while true
      |         u = rand(1);
      | 	    x = (alpha - log((1.0 - u)/u))/beta;
      | 	    n = floor(x + 0.5);
      | 	    if (n < 0)
      | 		    continue;
      |         end    
      | 	    v = rand(1);
      | 	    y = alpha - beta*x;
      | 	    lhs = y + log(v/(1.0 + exp(y))^2);
      | 	    rhs = k + n*log(lambda) - log(factorial(n));
      | 	    if (lhs <= rhs)
      | 		    break;
      |         end    
      |     end  
      |     dt = n / serviceRate;
      settings: OutputPortMap=o4,o5,o9
  Entity Server23 : EntityServer  InputPortMessageModes=m  OutputPortMessageModes=n,n,m  Capacity=1  ServiceTimeSource=MATLAB action  ServiceTimeValue=20  ServiceTimeAttributeName=entity.ServiceTime  ServiceTimeAction=|  AverageWait=on  Utilization=on
      | c = 0.767 - 3.36/lambda;
      |     beta = pi/sqrt(3.0*lambda);
      |     alpha = beta*lambda;
      |     k = log(c) - lambda - log(beta);
      | 
      |     while true
      |         u = rand(1);
      | 	    x = (alpha - log((1.0 - u)/u))/beta;
      | 	    n = floor(x + 0.5);
      | 	    if (n < 0)
      | 		    continue;
      |         end    
      | 	    v = rand(1);
      | 	    y = alpha - beta*x;
      | 	    lhs = y + log(v/(1.0 + exp(y))^2);
      | 	    rhs = k + n*log(lambda) - log(factorial(n));
      | 	    if (lhs <= rhs)
      | 		    break;
      |         end    
      |     end  
      |     dt = n / serviceRate;
      settings: OutputPortMap=o4,o5,o9
  Entity Server24 : EntityServer  InputPortMessageModes=m  OutputPortMessageModes=n,n,m  Capacity=1  ServiceTimeSource=MATLAB action  ServiceTimeValue=20  ServiceTimeAttributeName=entity.ServiceTime  ServiceTimeAction=|  AverageWait=on  Utilization=on
      | c = 0.767 - 3.36/lambda;
      |     beta = pi/sqrt(3.0*lambda);
      |     alpha = beta*lambda;
      |     k = log(c) - lambda - log(beta);
      | 
      |     while true
      |         u = rand(1);
      | 	    x = (alpha - log((1.0 - u)/u))/beta;
      | 	    n = floor(x + 0.5);
      | 	    if (n < 0)
      | 		    continue;
      |         end    
      | 	    v = rand(1);
      | 	    y = alpha - beta*x;
      | 	    lhs = y + log(v/(1.0 + exp(y))^2);
      | 	    rhs = k + n*log(lambda) - log(factorial(n));
      | 	    if (lhs <= rhs)
      | 		    break;
      |         end    
      |     end  
      |     dt = n / serviceRate;
      settings: OutputPortMap=o4,o5,o9
  Entity Server25 : EntityServer  InputPortMessageModes=m  OutputPortMessageModes=n,n,m  Capacity=1  ServiceTimeSource=MATLAB action  ServiceTimeValue=20  ServiceTimeAttributeName=entity.ServiceTime  ServiceTimeAction=|  AverageWait=on  Utilization=on
      | c = 0.767 - 3.36/lambda;
      |     beta = pi/sqrt(3.0*lambda);
      |     alpha = beta*lambda;
      |     k = log(c) - lambda - log(beta);
      | 
      |     while true
      |         u = rand(1);
      | 	    x = (alpha - log((1.0 - u)/u))/beta;
      | 	    n = floor(x + 0.5);
      | 	    if (n < 0)
      | 		    continue;
      |         end    
      | 	    v = rand(1);
      | 	    y = alpha - beta*x;
      | 	    lhs = y + log(v/(1.0 + exp(y))^2);
      | 	    rhs = k + n*log(lambda) - log(factorial(n));
      | 	    if (lhs <= rhs)
      | 		    break;
      |         end    
      |     end  
      |     dt = n / serviceRate;
      settings: OutputPortMap=o4,o5,o9
  Entity Server26 : EntityServer  InputPortMessageModes=m  OutputPortMessageModes=n,n,m  Capacity=1  ServiceTimeSource=MATLAB action  ServiceTimeValue=20  ServiceTimeAttributeName=entity.ServiceTime  ServiceTimeAction=|  AverageWait=on  Utilization=on
      | c = 0.767 - 3.36/lambda;
      |     beta = pi/sqrt(3.0*lambda);
      |     alpha = beta*lambda;
      |     k = log(c) - lambda - log(beta);
      | 
      |     while true
      |         u = rand(1);
      | 	    x = (alpha - log((1.0 - u)/u))/beta;
      | 	    n = floor(x + 0.5);
      | 	    if (n < 0)
      | 		    continue;
      |         end    
      | 	    v = rand(1);
      | 	    y = alpha - beta*x;
      | 	    lhs = y + log(v/(1.0 + exp(y))^2);
      | 	    rhs = k + n*log(lambda) - log(factorial(n));
      | 	    if (lhs <= rhs)
      | 		    break;
      |         end    
      |     end  
      |     dt = n / serviceRate;
      settings: OutputPortMap=o4,o5,o9
  Entity Server27 : EntityServer  InputPortMessageModes=m  OutputPortMessageModes=n,n,m  Capacity=1  ServiceTimeSource=MATLAB action  ServiceTimeValue=20  ServiceTimeAttributeName=entity.ServiceTime  ServiceTimeAction=|  AverageWait=on  Utilization=on
      | c = 0.767 - 3.36/lambda;
      |     beta = pi/sqrt(3.0*lambda);
      |     alpha = beta*lambda;
      |     k = log(c) - lambda - log(beta);
      | 
      |     while true
      |         u = rand(1);
      | 	    x = (alpha - log((1.0 - u)/u))/beta;
      | 	    n = floor(x + 0.5);
      | 	    if (n < 0)
      | 		    continue;
      |         end    
      | 	    v = rand(1);
      | 	    y = alpha - beta*x;
      | 	    lhs = y + log(v/(1.0 + exp(y))^2);
      | 	    rhs = k + n*log(lambda) - log(factorial(n));
      | 	    if (lhs <= rhs)
      | 		    break;
      |         end    
      |     end  
      |     dt = n / serviceRate;
      settings: OutputPortMap=o4,o5,o9
  Entity Server28 : EntityServer  InputPortMessageModes=m  OutputPortMessageModes=n,n,m  Capacity=1  ServiceTimeSource=MATLAB action  ServiceTimeValue=20  ServiceTimeAttributeName=entity.ServiceTime  ServiceTimeAction=|  AverageWait=on  Utilization=on
      | c = 0.767 - 3.36/lambda;
      |     beta = pi/sqrt(3.0*lambda);
      |     alpha = beta*lambda;
      |     k = log(c) - lambda - log(beta);
      | 
      |     while true
      |         u = rand(1);
      | 	    x = (alpha - log((1.0 - u)/u))/beta;
      | 	    n = floor(x + 0.5);
      | 	    if (n < 0)
      | 		    continue;
      |         end    
      | 	    v = rand(1);
      | 	    y = alpha - beta*x;
      | 	    lhs = y + log(v/(1.0 + exp(y))^2);
      | 	    rhs = k + n*log(lambda) - log(factorial(n));
      | 	    if (lhs <= rhs)
      | 		    break;
      |         end    
      |     end  
      |     dt = n / serviceRate;
      settings: OutputPortMap=o4,o5,o9
  Entity Server29 : EntityServer  InputPortMessageModes=m  OutputPortMessageModes=n,n,m  Capacity=1  ServiceTimeSource=MATLAB action  ServiceTimeValue=20  ServiceTimeAttributeName=entity.ServiceTime  ServiceTimeAction=|  AverageWait=on  Utilization=on
      | c = 0.767 - 3.36/lambda;
      |     beta = pi/sqrt(3.0*lambda);
      |     alpha = beta*lambda;
      |     k = log(c) - lambda - log(beta);
      | 
      |     while true
      |         u = rand(1);
      | 	    x = (alpha - log((1.0 - u)/u))/beta;
      | 	    n = floor(x + 0.5);
      | 	    if (n < 0)
      | 		    continue;
      |         end    
      | 	    v = rand(1);
      | 	    y = alpha - beta*x;
      | 	    lhs = y + log(v/(1.0 + exp(y))^2);
      | 	    rhs = k + n*log(lambda) - log(factorial(n));
      | 	    if (lhs <= rhs)
      | 		    break;
      |         end    
      |     end  
      |     dt = n / serviceRate;
      settings: OutputPortMap=o4,o5,o9
  Entity Server3 : EntityServer  InputPortMessageModes=m  OutputPortMessageModes=n,n,m  Capacity=1  ServiceTimeSource=MATLAB action  ServiceTimeValue=20  ServiceTimeAttributeName=entity.ServiceTime  ServiceTimeAction=|  AverageWait=on  Utilization=on
      | c = 0.767 - 3.36/lambda;
      |     beta = pi/sqrt(3.0*lambda);
      |     alpha = beta*lambda;
      |     k = log(c) - lambda - log(beta);
      | 
      |     while true
      |         u = rand(1);
      | 	    x = (alpha - log((1.0 - u)/u))/beta;
      | 	    n = floor(x + 0.5);
      | 	    if (n < 0)
      | 		    continue;
      |         end    
      | 	    v = rand(1);
      | 	    y = alpha - beta*x;
      | 	    lhs = y + log(v/(1.0 + exp(y))^2);
      | 	    rhs = k + n*log(lambda) - log(factorial(n));
      | 	    if (lhs <= rhs)
      | 		    break;
      |         end    
      |     end  
      |     dt = n / serviceRate;
      settings: OutputPortMap=o4,o5,o9
  Entity Server30 : EntityServer  InputPortMessageModes=m  OutputPortMessageModes=n,n,m  Capacity=1  ServiceTimeSource=MATLAB action  ServiceTimeValue=20  ServiceTimeAttributeName=entity.ServiceTime  ServiceTimeAction=|  AverageWait=on  Utilization=on
      | c = 0.767 - 3.36/lambda;
      |     beta = pi/sqrt(3.0*lambda);
      |     alpha = beta*lambda;
      |     k = log(c) - lambda - log(beta);
      | 
      |     while true
      |         u = rand(1);
      | 	    x = (alpha - log((1.0 - u)/u))/beta;
      | 	    n = floor(x + 0.5);
      | 	    if (n < 0)
      | 		    continue;
      |         end    
      | 	    v = rand(1);
      | 	    y = alpha - beta*x;
      | 	    lhs = y + log(v/(1.0 + exp(y))^2);
      | 	    rhs = k + n*log(lambda) - log(factorial(n));
      | 	    if (lhs <= rhs)
      | 		    break;
      |         end    
      |     end  
      |     dt = n / serviceRate;
      settings: OutputPortMap=o4,o5,o9
  Entity Server31 : EntityServer  InputPortMessageModes=m  OutputPortMessageModes=n,n,m  Capacity=1  ServiceTimeSource=MATLAB action  ServiceTimeValue=20  ServiceTimeAttributeName=entity.ServiceTime  ServiceTimeAction=|  AverageWait=on  Utilization=on
      | c = 0.767 - 3.36/lambda;
      |     beta = pi/sqrt(3.0*lambda);
      |     alpha = beta*lambda;
      |     k = log(c) - lambda - log(beta);
      | 
      |     while true
      |         u = rand(1);
      | 	    x = (alpha - log((1.0 - u)/u))/beta;
      | 	    n = floor(x + 0.5);
      | 	    if (n < 0)
      | 		    continue;
      |         end    
      | 	    v = rand(1);
      | 	    y = alpha - beta*x;
      | 	    lhs = y + log(v/(1.0 + exp(y))^2);
      | 	    rhs = k + n*log(lambda) - log(factorial(n));
      | 	    if (lhs <= rhs)
      | 		    break;
      |         end    
      |     end  
      |     dt = n / serviceRate;
      settings: OutputPortMap=o4,o5,o9
  Entity Server32 : EntityServer  InputPortMessageModes=m  OutputPortMessageModes=n,n,m  Capacity=1  ServiceTimeSource=MATLAB action  ServiceTimeValue=20  ServiceTimeAttributeName=entity.ServiceTime  ServiceTimeAction=|  AverageWait=on  Utilization=on
      | c = 0.767 - 3.36/lambda;
      |     beta = pi/sqrt(3.0*lambda);
      |     alpha = beta*lambda;
      |     k = log(c) - lambda - log(beta);
      | 
      |     while true
      |         u = rand(1);
      | 	    x = (alpha - log((1.0 - u)/u))/beta;
      | 	    n = floor(x + 0.5);
      | 	    if (n < 0)
      | 		    continue;
      |         end    
      | 	    v = rand(1);
      | 	    y = alpha - beta*x;
      | 	    lhs = y + log(v/(1.0 + exp(y))^2);
      | 	    rhs = k + n*log(lambda) - log(factorial(n));
      | 	    if (lhs <= rhs)
      | 		    break;
      |         end    
      |     end  
      |     dt = n / serviceRate;
      settings: OutputPortMap=o4,o5,o9
  Entity Server33 : EntityServer  InputPortMessageModes=m  OutputPortMessageModes=n,n,m  Capacity=1  ServiceTimeSource=MATLAB action  ServiceTimeValue=20  ServiceTimeAttributeName=entity.ServiceTime  ServiceTimeAction=|  AverageWait=on  Utilization=on
      | c = 0.767 - 3.36/lambda;
      |     beta = pi/sqrt(3.0*lambda);
      |     alpha = beta*lambda;
      |     k = log(c) - lambda - log(beta);
      | 
      |     while true
      |         u = rand(1);
      | 	    x = (alpha - log((1.0 - u)/u))/beta;
      | 	    n = floor(x + 0.5);
      | 	    if (n < 0)
      | 		    continue;
      |         end    
      | 	    v = rand(1);
      | 	    y = alpha - beta*x;
      | 	    lhs = y + log(v/(1.0 + exp(y))^2);
      | 	    rhs = k + n*log(lambda) - log(factorial(n));
      | 	    if (lhs <= rhs)
      | 		    break;
      |         end    
      |     end  
      |     dt = n / serviceRate;
      settings: OutputPortMap=o4,o5,o9
  Entity Server34 : EntityServer  InputPortMessageModes=m  OutputPortMessageModes=n,n,m  Capacity=1  ServiceTimeSource=MATLAB action  ServiceTimeValue=20  ServiceTimeAttributeName=entity.ServiceTime  ServiceTimeAction=|  AverageWait=on  Utilization=on
      | c = 0.767 - 3.36/lambda;
      |     beta = pi/sqrt(3.0*lambda);
      |     alpha = beta*lambda;
      |     k = log(c) - lambda - log(beta);
      | 
      |     while true
      |         u = rand(1);
      | 	    x = (alpha - log((1.0 - u)/u))/beta;
      | 	    n = floor(x + 0.5);
      | 	    if (n < 0)
      | 		    continue;
      |         end    
      | 	    v = rand(1);
      | 	    y = alpha - beta*x;
      | 	    lhs = y + log(v/(1.0 + exp(y))^2);
      | 	    rhs = k + n*log(lambda) - log(factorial(n));
      | 	    if (lhs <= rhs)
      | 		    break;
      |         end    
      |     end  
      |     dt = n / serviceRate;
      settings: OutputPortMap=o4,o5,o9
  Entity Server4 : EntityServer  InputPortMessageModes=m  OutputPortMessageModes=n,n,m  Capacity=1  ServiceTimeSource=MATLAB action  ServiceTimeValue=20  ServiceTimeAttributeName=entity.ServiceTime  ServiceTimeAction=|  AverageWait=on  Utilization=on
      | c = 0.767 - 3.36/lambda;
      |     beta = pi/sqrt(3.0*lambda);
      |     alpha = beta*lambda;
      |     k = log(c) - lambda - log(beta);
      | 
      |     while true
      |         u = rand(1);
      | 	    x = (alpha - log((1.0 - u)/u))/beta;
      | 	    n = floor(x + 0.5);
      | 	    if (n < 0)
      | 		    continue;
      |         end    
      | 	    v = rand(1);
      | 	    y = alpha - beta*x;
      | 	    lhs = y + log(v/(1.0 + exp(y))^2);
      | 	    rhs = k + n*log(lambda) - log(factorial(n));
      | 	    if (lhs <= rhs)
      | 		    break;
      |         end    
      |     end  
      |     dt = n / serviceRate;
      settings: OutputPortMap=o4,o5,o9
  Entity Server5 : EntityServer  InputPortMessageModes=m  OutputPortMessageModes=n,n,m  Capacity=1  ServiceTimeSource=MATLAB action  ServiceTimeValue=20  ServiceTimeAttributeName=entity.ServiceTime  ServiceTimeAction=|  AverageWait=on  Utilization=on
      | c = 0.767 - 3.36/lambda;
      |     beta = pi/sqrt(3.0*lambda);
      |     alpha = beta*lambda;
      |     k = log(c) - lambda - log(beta);
      | 
      |     while true
      |         u = rand(1);
      | 	    x = (alpha - log((1.0 - u)/u))/beta;
      | 	    n = floor(x + 0.5);
      | 	    if (n < 0)
      | 		    continue;
      |         end    
      | 	    v = rand(1);
      | 	    y = alpha - beta*x;
      | 	    lhs = y + log(v/(1.0 + exp(y))^2);
      | 	    rhs = k + n*log(lambda) - log(factorial(n));
      | 	    if (lhs <= rhs)
      | 		    break;
      |         end    
      |     end  
      |     dt = n / serviceRate;
      settings: OutputPortMap=o4,o5,o9
  Entity Server6 : EntityServer  InputPortMessageModes=m  OutputPortMessageModes=n,n,m  Capacity=1  ServiceTimeSource=MATLAB action  ServiceTimeValue=20  ServiceTimeAttributeName=entity.ServiceTime  ServiceTimeAction=|  AverageWait=on  Utilization=on
      | c = 0.767 - 3.36/lambda;
      |     beta = pi/sqrt(3.0*lambda);
      |     alpha = beta*lambda;
      |     k = log(c) - lambda - log(beta);
      | 
      |     while true
      |         u = rand(1);
      | 	    x = (alpha - log((1.0 - u)/u))/beta;
      | 	    n = floor(x + 0.5);
      | 	    if (n < 0)
      | 		    continue;
      |         end    
      | 	    v = rand(1);
      | 	    y = alpha - beta*x;
      | 	    lhs = y + log(v/(1.0 + exp(y))^2);
      | 	    rhs = k + n*log(lambda) - log(factorial(n));
      | 	    if (lhs <= rhs)
      | 		    break;
      |         end    
      |     end  
      |     dt = n / serviceRate;
      settings: OutputPortMap=o4,o5,o9
  Entity Server7 : EntityServer  InputPortMessageModes=m  OutputPortMessageModes=n,n,m  Capacity=1  ServiceTimeSource=MATLAB action  ServiceTimeValue=20  ServiceTimeAttributeName=entity.ServiceTime  ServiceTimeAction=|  AverageWait=on  Utilization=on
      | c = 0.767 - 3.36/lambda;
      |     beta = pi/sqrt(3.0*lambda);
      |     alpha = beta*lambda;
      |     k = log(c) - lambda - log(beta);
      | 
      |     while true
      |         u = rand(1);
      | 	    x = (alpha - log((1.0 - u)/u))/beta;
      | 	    n = floor(x + 0.5);
      | 	    if (n < 0)
      | 		    continue;
      |         end    
      | 	    v = rand(1);
      | 	    y = alpha - beta*x;
      | 	    lhs = y + log(v/(1.0 + exp(y))^2);
      | 	    rhs = k + n*log(lambda) - log(factorial(n));
      | 	    if (lhs <= rhs)
      | 		    break;
      |         end    
      |     end  
      |     dt = n  / serviceRate;
      settings: OutputPortMap=o4,o5,o9
  Entity Server8 : EntityServer  InputPortMessageModes=m  OutputPortMessageModes=n,n,m  Capacity=1  ServiceTimeSource=MATLAB action  ServiceTimeValue=20  ServiceTimeAttributeName=entity.ServiceTime  ServiceTimeAction=|  AverageWait=on  Utilization=on
      | c = 0.767 - 3.36/lambda;
      |     beta = pi/sqrt(3.0*lambda);
      |     alpha = beta*lambda;
      |     k = log(c) - lambda - log(beta);
      | 
      |     while true
      |         u = rand(1);
      | 	    x = (alpha - log((1.0 - u)/u))/beta;
      | 	    n = floor(x + 0.5);
      | 	    if (n < 0)
      | 		    continue;
      |         end    
      | 	    v = rand(1);
      | 	    y = alpha - beta*x;
      | 	    lhs = y + log(v/(1.0 + exp(y))^2);
      | 	    rhs = k + n*log(lambda) - log(factorial(n));
      | 	    if (lhs <= rhs)
      | 		    break;
      |         end    
      |     end  
      |     dt = n / serviceRate;
      settings: OutputPortMap=o4,o5,o9
  Entity Server9 : EntityServer  InputPortMessageModes=m  OutputPortMessageModes=n,n,m  Capacity=1  ServiceTimeSource=MATLAB action  ServiceTimeValue=20  ServiceTimeAttributeName=entity.ServiceTime  ServiceTimeAction=|  AverageWait=on  Utilization=on
      | c = 0.767 - 3.36/lambda;
      |     beta = pi/sqrt(3.0*lambda);
      |     alpha = beta*lambda;
      |     k = log(c) - lambda - log(beta);
      | 
      |     while true
      |         u = rand(1);
      | 	    x = (alpha - log((1.0 - u)/u))/beta;
      | 	    n = floor(x + 0.5);
      | 	    if (n < 0)
      | 		    continue;
      |         end    
      | 	    v = rand(1);
      | 	    y = alpha - beta*x;
      | 	    lhs = y + log(v/(1.0 + exp(y))^2);
      | 	    rhs = k + n*log(lambda) - log(factorial(n));
      | 	    if (lhs <= rhs)
      | 		    break;
      |         end    
      |     end  
      |     dt = n / serviceRate;
      settings: OutputPortMap=o4,o5,o9
  Entity Terminator{,1..34} (35 alike) : EntityTerminator  InputPortMessageModes=m
  Gain : Gain  Gain=100
  Gain1 : Gain  Gain=31
  MATLAB Function : MATLAB Function  TreatAsAtomicUnit=on
  Scope : Scope
  Scope5 : Scope
  Sum : Sum  Inputs=+++++++++++++++++++++++++++++++++++
  Sum1 : Sum  Inputs=+++++++++++++++++++++++++++++++++++
  Switch : Switch  Threshold=scalingLoopDelay
  Switch1 : Switch  Threshold=initialLoopWaitTime
  Vector Concatenate : Concatenate  NumInputs=35
  Vector Concatenate1 : Concatenate  NumInputs=35
  Cores : Outport
  utilPerCore : Outport  Port=2
  outDelay : Outport  Port=3
  utilOf1 : Outport  Port=4
  waitOf1 : Outport  Port=5
  wires:
  Entity Server1/3 -> Entity Terminator1/1
  Entity Server/3 -> Entity Terminator/1
  Entity Output Switch/3 -> Blocker3/1(In1)
  Entity Output Switch/4 -> Blocker4/1(In1)
  Gain1/1 -> Cores/1, Divide1/2, Divide/2, Core controller/1(In1), MATLAB Function/5(coresNow)
  Entity Server4/2 -> Sum/2
  Entity Server3/3 -> Entity Terminator3/1
  Core controller/2(Out2) -> Vector Concatenate/2, Blocker2/2(control)
  Entity Output Switch/1 -> Blocker1/1(In1)
  Entity Server1/2 -> Sum/5
  Entity Server/2 -> utilOf1/1, Sum/1
  Entity Output Switch/2 -> Blocker2/1(In1)
  Entity Server3/2 -> Sum/3
  Entity Output Switch/5 -> Blocker5/1(In1)
  Core controller/3(Out3) -> Vector Concatenate/3, Blocker3/2(control)
  Entity Server2/3 -> Entity Terminator2/1
  Entity Server2/2 -> Sum/4
  Entity Server4/3 -> Entity Terminator4/1
  In1/1 -> Entity Output Switch/2
  Sum/1 -> Gain/1
  Core controller/1(control) -> Blocker1/2(control), Vector Concatenate/1
  Constant1/1 -> MATLAB Function/3(maxCores)
  Core controller/4(Out4) -> Vector Concatenate/4, Blocker4/2(control)
  Constant/1 -> Gain1/1
  Core controller/5(Out5) -> Vector Concatenate/5, Blocker5/2(control)
  Constant3/1 -> MATLAB Function/1(upperThresh)
  Constant2/1 -> MATLAB Function/2(lowerThresh)
  Entity Server5/3 -> Entity Terminator5/1
  Entity Output Switch/6 -> Blocker6/1(In1)
  Entity Server6/3 -> Entity Terminator6/1
  Entity Output Switch/7 -> Blocker7/1(In1)
  Entity Server7/3 -> Entity Terminator7/1
  Entity Output Switch/8 -> Blocker8/1(In1)
  Entity Server8/3 -> Entity Terminator8/1
  Entity Server9/3 -> Entity Terminator9/1
  Entity Output Switch/10 -> Blocker9/1(In1)
  Entity Server10/3 -> Entity Terminator10/1
  Entity Output Switch/11 -> Blocker10/1(In1)
  Entity Server11/3 -> Entity Terminator11/1
  Entity Output Switch/12 -> Blocker11/1(In1)
  Entity Server12/3 -> Entity Terminator12/1
  Entity Output Switch/13 -> Blocker12/1(In1)
  Entity Server13/3 -> Entity Terminator13/1
  Entity Output Switch/14 -> Blocker13/1(In1)
  Entity Server14/3 -> Entity Terminator14/1
  Entity Output Switch/15 -> Blocker14/1(In1)
  Entity Server15/3 -> Entity Terminator15/1
  Entity Output Switch/16 -> Blocker15/1(In1)
  Entity Server16/3 -> Entity Terminator16/1
  Entity Output Switch/17 -> Blocker16/1(In1)
  Entity Server17/3 -> Entity Terminator17/1
  Entity Output Switch/18 -> Blocker17/1(In1)
  Entity Server18/3 -> Entity Terminator18/1
  Entity Output Switch/19 -> Blocker18/1(In1)
  Entity Server19/3 -> Entity Terminator19/1
  Entity Output Switch/20 -> Blocker19/1(In1)
  Entity Server20/3 -> Entity Terminator20/1
  Entity Output Switch/21 -> Blocker20/1(In1)
  Entity Server21/3 -> Entity Terminator21/1
  Entity Output Switch/22 -> Blocker21/1(In1)
  Entity Server22/3 -> Entity Terminator22/1
  Entity Output Switch/23 -> Blocker22/1(In1)
  Entity Server23/3 -> Entity Terminator23/1
  Entity Output Switch/24 -> Blocker23/1(In1)
  Entity Server24/3 -> Entity Terminator24/1
  Entity Output Switch/25 -> Blocker24/1(In1)
  Entity Server25/3 -> Entity Terminator25/1
  Entity Output Switch/26 -> Blocker25/1(In1)
  Entity Server26/3 -> Entity Terminator26/1
  Entity Output Switch/27 -> Blocker26/1(In1)
  Entity Server27/3 -> Entity Terminator27/1
  Entity Output Switch/28 -> Blocker27/1(In1)
  Entity Server28/3 -> Entity Terminator28/1
  Entity Output Switch/29 -> Blocker28/1(In1)
  Entity Server29/3 -> Entity Terminator29/1
  Entity Output Switch/30 -> Blocker29/1(In1)
  Entity Server30/3 -> Entity Terminator30/1
  Entity Output Switch/31 -> Blocker30/1(In1)
  Entity Server31/3 -> Entity Terminator31/1
  Entity Output Switch/32 -> Blocker31/1(In1)
  Entity Server32/3 -> Entity Terminator32/1
  Entity Output Switch/33 -> Blocker32/1(In1)
  Entity Server33/3 -> Entity Terminator33/1
  Entity Output Switch/34 -> Blocker33/1(In1)
  Entity Server34/3 -> Entity Terminator34/1
  Entity Output Switch/35 -> Blocker34/1(In1)
  Entity Server5/2 -> Sum/6
  Entity Server6/2 -> Sum/7
  Entity Server7/2 -> Sum/8
  Entity Server8/2 -> Sum/9
  Entity Server9/2 -> Sum/10
  Entity Server10/2 -> Scope5/1, Sum/11
  Entity Server11/2 -> Sum/12
  Entity Server12/2 -> Sum/13
  Entity Server13/2 -> Sum/14
  Entity Server14/2 -> Sum/15
  Entity Server15/2 -> Sum/16
  Entity Server16/2 -> Sum/17
  Entity Server17/2 -> Sum/18
  Entity Server18/2 -> Sum/19
  Entity Server19/2 -> Sum/20
  Entity Server20/2 -> Sum/21
  Entity Server21/2 -> Sum/22
  Entity Server22/2 -> Sum/23
  Entity Server23/2 -> Sum/24
  Entity Server24/2 -> Sum/25
  Entity Server25/2 -> Sum/26
  Entity Server26/2 -> Sum/27
  Entity Server27/2 -> Sum/28
  Entity Server28/2 -> Sum/29
  Entity Server29/2 -> Sum/30
  Entity Server30/2 -> Sum/31
  Entity Server31/2 -> Sum/32
  Entity Server32/2 -> Sum/33
  Entity Server33/2 -> Sum/34
  Entity Server34/2 -> Sum/35
  Core controller/6(Out6) -> Vector Concatenate/6, Blocker6/2(control)
  Core controller/7(Out7) -> Vector Concatenate/7, Blocker7/2(control)
  Core controller/9(Out9) -> Vector Concatenate/9, Blocker/2(control)
  Core controller/10(Out10) -> Vector Concatenate/10, Blocker9/2(control)
  Core controller/11(Out11) -> Vector Concatenate/11, Blocker10/2(control)
  Core controller/12(Out12) -> Vector Concatenate/12, Blocker11/2(control)
  Core controller/13(Out13) -> Vector Concatenate/13, Blocker12/2(control)
  Core controller/15(Out15) -> Vector Concatenate/15, Blocker14/2(control)
  Core controller/16(Out16) -> Vector Concatenate/16, Blocker15/2(control)
  Core controller/17(Out17) -> Blocker16/2(control), Vector Concatenate/17
  Core controller/18(Out18) -> Blocker17/2(control), Vector Concatenate/18
  Core controller/19(Out19) -> Vector Concatenate/19, Blocker18/2(control)
  Core controller/20(Out20) -> Vector Concatenate/20, Blocker19/2(control)
  Core controller/21(Out21) -> Blocker20/2(control), Vector Concatenate/21
  Core controller/22(Out22) -> Vector Concatenate/22, Blocker21/2(control)
  Core controller/23(Out23) -> Vector Concatenate/23, Blocker22/2(control)
  Core controller/24(Out24) -> Blocker23/2(control), Vector Concatenate/24
  Core controller/25(Out25) -> Vector Concatenate/25, Blocker24/2(control)
  Core controller/26(Out26) -> Blocker25/2(control), Vector Concatenate/26
  Core controller/27(Out27) -> Vector Concatenate/27, Blocker26/2(control)
  Core controller/28(Out28) -> Vector Concatenate/28, Blocker27/2(control)
  Core controller/29(Out29) -> Vector Concatenate/29, Blocker28/2(control)
  Core controller/30(Out30) -> Vector Concatenate/30, Blocker29/2(control)
  Core controller/31(Out31) -> Vector Concatenate/31, Blocker30/2(control)
  Core controller/32(Out32) -> Vector Concatenate/32, Blocker31/2(control)
  Core controller/33(Out33) -> Vector Concatenate/33, Blocker32/2(control)
  Core controller/34(Out34) -> Vector Concatenate/34, Blocker33/2(control)
  Core controller/35(Out35) -> Vector Concatenate/35, Blocker34/2(control)
  Counter Limited/1 -> Switch/2
  Constant4/1 -> Switch1/3, Switch/3
  Switch/1 -> MATLAB Function/6(util)
  Gain/1 -> Scope/1, Switch1/1, Divide/1
  Divide/1 -> utilPerCore/1
  Counter Free-Running/1 -> Switch1/2
  Switch1/1 -> Switch/1
  Entity Output Switch/9 -> Blocker/1(In1)
  Blocker/1(Out1) -> Entity Queue8/1
  Blocker1/1(Out1) -> Entity Queue/1
  Blocker2/1(Out1) -> Entity Queue1/1
  Blocker3/1(Out1) -> Entity Queue2/1
  Blocker4/1(Out1) -> Entity Queue3/1
  Blocker5/1(Out1) -> Entity Queue4/1
  Blocker6/1(Out1) -> Entity Queue5/1
  Blocker7/1(Out1) -> Entity Queue6/1
  Blocker8/1(Out1) -> Entity Queue7/1
  Blocker9/1(Out1) -> Entity Queue9/1
  Blocker10/1(Out1) -> Entity Queue10/1
  Blocker11/1(Out1) -> Entity Queue11/1
  Blocker12/1(Out1) -> Entity Queue12/1
  Blocker13/1(Out1) -> Entity Queue13/1
  Blocker14/1(Out1) -> Entity Queue14/1
  Blocker15/1(Out1) -> Entity Queue15/1
  Blocker16/1(Out1) -> Entity Queue16/1
  Blocker17/1(Out1) -> Entity Queue17/1
  Blocker18/1(Out1) -> Entity Queue18/1
  Blocker19/1(Out1) -> Entity Queue19/1
  Blocker20/1(Out1) -> Entity Queue20/1
  Blocker21/1(Out1) -> Entity Queue21/1
  Blocker22/1(Out1) -> Entity Queue22/1
  Blocker23/1(Out1) -> Entity Queue23/1
  Blocker24/1(Out1) -> Entity Queue24/1
  Blocker25/1(Out1) -> Entity Queue25/1
  Blocker26/1(Out1) -> Entity Queue26/1
  Blocker27/1(Out1) -> Entity Queue27/1
  Blocker28/1(Out1) -> Entity Queue28/1
  Blocker29/1(Out1) -> Entity Queue29/1
  Blocker30/1(Out1) -> Entity Queue30/1
  Blocker31/1(Out1) -> Entity Queue31/1
  Blocker32/1(Out1) -> Entity Queue32/1
  Blocker33/1(Out1) -> Entity Queue33/1
  Blocker34/1(Out1) -> Entity Queue34/1
  Constant5/1 -> MATLAB Function/4(scalingStep)
  Entity Queue/3 -> Entity Server/1
  Entity Queue1/3 -> Entity Server4/1
  Entity Queue2/3 -> Entity Server3/1
  Entity Queue3/3 -> Entity Server2/1
  Entity Queue4/3 -> Entity Server1/1
  Entity Queue5/3 -> Entity Server5/1
  Entity Queue6/3 -> Entity Server6/1
  Entity Queue7/3 -> Entity Server7/1
  Entity Queue8/3 -> Entity Server8/1
  Entity Queue9/3 -> Entity Server9/1
  Entity Queue10/3 -> Entity Server10/1
  Entity Queue11/3 -> Entity Server11/1
  Entity Queue12/3 -> Entity Server12/1
  Entity Queue13/3 -> Entity Server13/1
  Entity Queue14/3 -> Entity Server14/1
  Entity Queue15/3 -> Entity Server15/1
  Entity Queue16/3 -> Entity Server16/1
  Entity Queue17/3 -> Entity Server17/1
  Entity Queue18/3 -> Entity Server18/1
  Entity Queue19/3 -> Entity Server19/1
  Entity Queue20/3 -> Entity Server20/1
  Entity Queue21/3 -> Entity Server21/1
  Entity Queue22/3 -> Entity Server22/1
  Entity Queue23/3 -> Entity Server23/1
  Entity Queue24/3 -> Entity Server24/1
  Entity Queue25/3 -> Entity Server25/1
  Entity Queue26/3 -> Entity Server26/1
  Entity Queue27/3 -> Entity Server27/1
  Entity Queue28/3 -> Entity Server28/1
  Entity Queue29/3 -> Entity Server29/1
  Entity Queue30/3 -> Entity Server30/1
  Entity Queue31/3 -> Entity Server31/1
  Entity Queue32/3 -> Entity Server32/1
  Entity Queue33/3 -> Entity Server33/1
  Entity Queue34/3 -> Entity Server34/1
  Core controller/8(Out8) -> Vector Concatenate/8, Blocker8/2(control)
  Core controller/14(Out14) -> Vector Concatenate/14, Blocker13/2(control)
  Entity Queue34/1 -> Vector Concatenate1/35
  Entity Queue33/1 -> Vector Concatenate1/34
  Entity Queue32/1 -> Vector Concatenate1/33
  Entity Queue31/1 -> Vector Concatenate1/32
  Entity Queue30/1 -> Vector Concatenate1/31
  Entity Queue29/1 -> Vector Concatenate1/30
  Entity Queue28/1 -> Vector Concatenate1/29
  Entity Queue27/1 -> Vector Concatenate1/28
  Entity Queue26/1 -> Vector Concatenate1/27
  Entity Queue25/1 -> Vector Concatenate1/26
  Entity Queue24/1 -> Vector Concatenate1/25
  Entity Queue23/1 -> Vector Concatenate1/24
  Entity Queue22/1 -> Vector Concatenate1/23
  Entity Queue21/1 -> Vector Concatenate1/22
  Entity Queue20/1 -> Vector Concatenate1/21
  Entity Queue19/1 -> Vector Concatenate1/20
  Entity Queue18/1 -> Vector Concatenate1/19
  Entity Queue17/1 -> Vector Concatenate1/18
  Entity Queue16/1 -> Vector Concatenate1/17
  Entity Queue15/1 -> Vector Concatenate1/16
  Entity Queue14/1 -> Vector Concatenate1/15
  Entity Queue13/1 -> Vector Concatenate1/14
  Entity Queue12/1 -> Vector Concatenate1/13
  Entity Queue11/1 -> Vector Concatenate1/12
  Entity Queue10/1 -> Vector Concatenate1/11
  Entity Queue9/1 -> Vector Concatenate1/10
  Entity Queue8/1 -> Vector Concatenate1/9
  Entity Queue7/1 -> Vector Concatenate1/8
  Entity Queue6/1 -> Vector Concatenate1/7
  Entity Queue5/1 -> Vector Concatenate1/6
  Entity Queue4/1 -> Vector Concatenate1/5
  Entity Queue3/1 -> Vector Concatenate1/4
  Entity Queue2/1 -> Vector Concatenate1/3
  Entity Queue1/1 -> Vector Concatenate1/2
  Entity Queue/1 -> Vector Concatenate1/1
  Vector Concatenate/1 -> Balancer/1(blocked)
  Vector Concatenate1/1 -> Balancer/2(fillOf)
  Balancer/1(SelectedPort) -> Entity Output Switch/1
  Entity Server/1 -> Sum1/1, waitOf1/1
  Entity Server4/1 -> Sum1/2
  Entity Server3/1 -> Sum1/3
  Entity Server2/1 -> Sum1/4
  Entity Server1/1 -> Sum1/5
  Entity Server5/1 -> Sum1/6
  Entity Server6/1 -> Sum1/7
  Entity Server7/1 -> Sum1/8
  Entity Server8/1 -> Sum1/9
  Entity Server9/1 -> Sum1/10
  Entity Server10/1 -> Sum1/11
  Entity Server11/1 -> Sum1/12
  Entity Server12/1 -> Sum1/13
  Entity Server13/1 -> Sum1/14
  Entity Server14/1 -> Sum1/15
  Entity Server15/1 -> Sum1/16
  Entity Server16/1 -> Sum1/17
  Entity Server17/1 -> Sum1/18
  Entity Server18/1 -> Sum1/19
  Entity Server19/1 -> Sum1/20
  Entity Server20/1 -> Sum1/21
  Entity Server21/1 -> Sum1/22
  Entity Server22/1 -> Sum1/23
  Entity Server23/1 -> Sum1/24
  Entity Server24/1 -> Sum1/25
  Entity Server25/1 -> Sum1/26
  Entity Server26/1 -> Sum1/27
  Entity Server27/1 -> Sum1/28
  Entity Server28/1 -> Sum1/29
  Entity Server29/1 -> Sum1/30
  Entity Server30/1 -> Sum1/31
  Entity Server31/1 -> Sum1/32
  Entity Server32/1 -> Sum1/33
  Entity Server33/1 -> Sum1/34
  Entity Server34/1 -> Sum1/35
  Sum1/1 -> Divide1/1
  Divide1/1 -> outDelay/1
